simulink model "dynamically_speed_controlled_dc_wound_motor_regen_braking"  (R2025a)
settings: Solver=ode15s  StartTime=0.0  StopTime=40  MaxStep=1e-4  RelTol=1e-3
undefined symbols (not defined in the file): Thyristor
libraries: fl_lib x13, nesl_utility x7, ee_lib x5
(part 1 of 2)
settings Model: Creator=User  LastModifiedBy=User
settings SolverCC: ZeroCrossAlgorithm=Adaptive

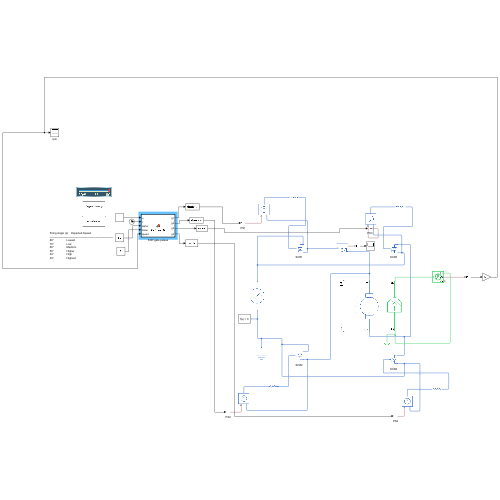
[thumbnail: Simulink's stored preview of the top-level diagram]
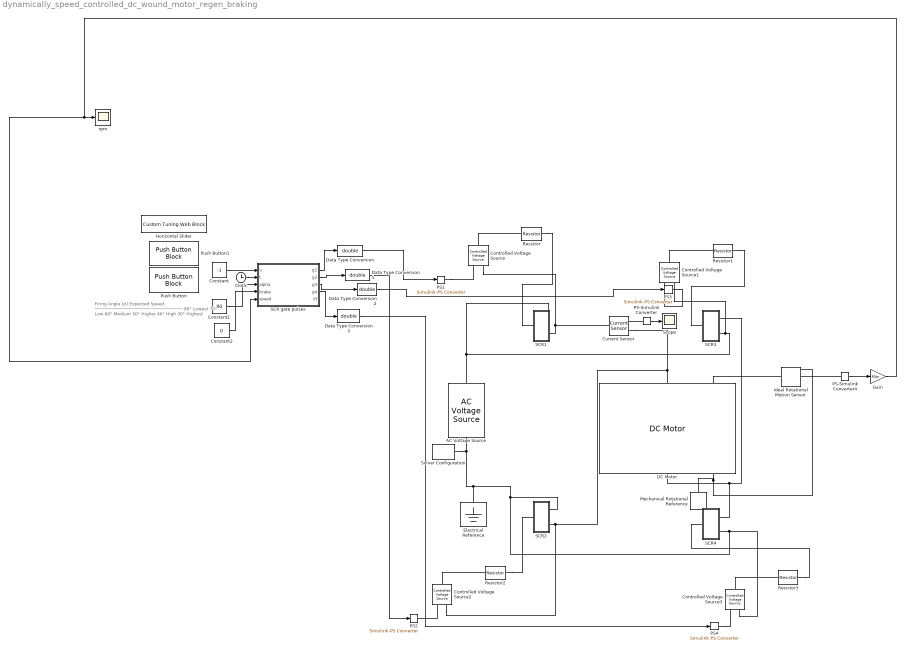
== system dynamically_speed_controlled_dc_wound_motor_regen_braking ==
  note: Firing Angle (α)    Expected Speed
      | ─────────────────────────────────
      | 80°                 Lowest
      | 70°                 Low
      | 60°                 Medium
      | 50°                 Higher
      | 40°                 High
      | 30°                 Highest
  AC Voltage Source : fl_lib/Electrical/Electrical Sources/AC Voltage Source  amp=100 V  shift=0 deg  frequency=50 Hz
  Clock : Clock
  Constant : Constant  Value=-1
  Constant1 : Constant  Value=80
  Constant2 : Constant  Value=0
  Controlled Voltage Source{,1..3} (4 alike) : fl_lib/Electrical/Electrical Sources/Controlled Voltage Source
  Current Sensor : fl_lib/Electrical/Electrical Sensors/Current Sensor
  DC Motor : ee_lib/Electromechanical/Brushed Motors/DC Motor  field_option=ee.enum.field_option.wound  Rf=100 Ohm  Lf=1 H  Laf=0.15 H  If0=0.24 A  parameterization=ee.enum.dcparam_option.circuit_param  Ra=3.9 Ohm  La="0.1  H"  emf_or_torque=ee.enum.emf_or_torque.kv  Kv=0.072e-3 V/rpm  Ki=6.876e-4 N*m/A  T_stall=0.24e-3 N*m  w_max=19100 rpm  w_rated=15000 rpm  P_rated=0.08 W  V_rated=1.5 V  lam_param=ee.enum.lam_param.damping  i_noload=0 A  V_i_noload=1.5 V  J=100 cm^2*g  lam=1e-5 N*m*s/rad  speed0=0 rpm  alpha=3.93e-3 1/K  Tmeas=25 degC  thermal_mass=100 J/K  initial_temperature=25 degC
      settings: InternalSimscapePortConfiguration="{\"Bottom\":[],\"Left\":[{\"id\":\"fp\",\"label\":\"F+\",\"type\":\"foundation.electrical.electrical\"},{\"id\":\"p\",\"label\":\"+\",\"type\":\"foundation.electrical.electrical\"},{\"id\":\"R\",\"label\":\"R\",\"type\":\"foundation.mechanical.rotational.rotational\"}],\"Right\":[{\"id\":\"fn\",\"label\":\"F-\",\"type\":\"foundation.electrical.electrical\"},{\"id\":\"n\",\"label\":\"-\",\"type\":\"foundation.electrical.electrical\"},{\"id\":\"C\",\"label\":\"C\",\"type\":\"foundation.mechanical.rotational.rotational\"}],\"Top\":[]}"
  Data Type Conversion{,1..3} (4 alike) : DataTypeConversion  OutDataTypeStr=double  SaturateOnIntegerOverflow=off  RndMeth=Floor
  Electrical Reference : fl_lib/Electrical/Electrical Elements/Electrical Reference
  Gain : Gain  Gain=30/pi
  Horizontal Slider : CustomTuningWebBlock  LabelPosition=Hide  ShowInitialText=on  Configuration="{\"components\":[{\"name\":\"LinearScaleComponent\",\"settings\":{\"bounds\":{\"max\":80,\"min\":30,\"tickInterval\":\"auto\"},\"internalTickHeightScaleFactor\":0.5,\"labelColor\":[255,255,200],\"labelFont\":{\"font\":\"Arial\",\"fontSize\":12},\"labelOffset\":0.05,\"labelTransparency\":1,\"needleImage\":{\"size\":[596,842],\"src\":\"data:image\\/svg+xml;base64,PD94bWwgdmVyc2lvbj0iMS4wIiBlbmNvZGluZz0idXRmLTgiPz4NCjwhLS0gR2VuZXJhdG9yOiBBZG9iZSBJbGx1c3RyYXRvciAyNS4wLjAsIFNWRyBFeHBvcnQgUGx1Zy1JbiAuIFNWRyBWZXJzaW9uOiA2LjAwIEJ1aWxkIDApICAtLT4NCjxzdmcgdmVyc2lvbj0iMS4xIg0KCSBpZD0ic3ZnOCIgeG1sbnM6Y2M9Imh0dHA6Ly9jcmVhdGl2ZWNvbW1vbnMub3JnL25zIyIgeG1sbnM6ZGM9Imh0dHA6Ly9wdXJsLm9yZy9kYy9lbGVtZW50cy8xLjEvIiB4bWxuczppbmtzY2FwZT0iaHR0cDovL3d3dy5pbmtzY2FwZS5vcmcvbmFtZXNw ...(+2420 chars)\",\"srcOrientation\":\"Right\"},\"needleOffset\":[-0.8044596912521441,-0.0642123287671233],\"needleSize\":{\"height\":0.4337797619047619,\"width\":0.07668067226890757},\"position\":[0.2829861111111111,0.04398634453781513,0.9196428571428571,0.6088789682539683],\"referencePoint\":\"auto\",\"scaleColors\":[],\"scaleColorsSize\":0.2,\"scaleDirection\":\"LR\",\"showLabels\":1,\"showMinorTicks\":0,\"showSpanLine\":1,\"showTicks\":1,\"tickColor\":[252,252,197],\"tickTransparency\":1,\"valueBarColor\":[0,114,189],\"valueBarOffset\":-0.27,\"valueBarSize\":0.1,\"valueBarTransparency\":1}},{\"name\":\"BackgroundImageComponent\",\"settings\":{\"image\":{\"size\":[380,101],\"src\":\"data:image\\/svg+xml;base64,PHN2ZyB4bWxucz0iaHR0cDovL3d3dy53My5vcmcvMjAwMC9zdmciIHhtbG5zOnhsaW5rPSJodHRwOi8vd3d3LnczLm9yZy8xOTk5L3hsaW5rIiB2aWV3Qm94PSIwIDAgMzgwIDEwMSI+PGRlZnM+PHN0eWxlPi5jbHMtMXtmaWxsOiMwMDJiNDI7fS5jbHMtMntmaWxsOiM0MjcwODI7fS5jbHMtM3tmaWxsOnVybCgjcmFkaWFsLWdyYWRpZW50KTt9LmNscy00e2ZpbGw6I2M4YzhjODtzdHJva2U6IzAwMDt9PC9zdHlsZT48cmFkaWFsR3JhZGllbnQgaWQ9InJhZGlhbC1ncmFkaWVudCIgY3g9IjE5MCIgY3k9IjUwLjUiIHI9IjI2OS4yMSIgZ3JhZGllbnRVbml0cz0idXNlclNwYWNlT25Vc2UiPjxzdG9wIG9mZnNldD0iMC4wMSIgc3RvcC1jb2xvcj0iIzNlNGY1OCIvPjxzdG9wIG9mZnNldD0iMC4wNiIgc3RvcC1jb2xvcj0iIzQ0NTc2MSIvPjxzdG9wIG9mZnNldD0iMC4xNSIgc3RvcC1jb2xvcj0iIzU1NmE3NiIvPjxzdG9wIG9mZnNldD0iMC4yNSIgc3RvcC1jb2xvcj0iIzZkODg5NSIvPjxzdG9wIG9mZnNldD0iMC4zOCIgc3RvcC1jb2xvcj0iIzhmYjJjMyIvPjxzdG9wIG9mZnNldD0iMC41MiIgc3RvcC1jb2xvcj0iI2I2ZTRmYSIvPjxzdG9wIG9mZnNldD0iMSIgc3RvcC1jb2xvcj0iIzE1NDY1NyIvPjwvcmFkaWFsR3JhZGllbnQ+PC9kZWZzPjxnIGlkPSJmcmFtZSI+PGcgaWQ9IkxheWVyXzIiIGRhdGEtbmFtZT0iTGF5ZXIgMiI+PGcgaWQ9IkxheWVyXzEtMiIgZGF0YS1uYW1lPSJMYXllciAxLTIiPjxyZWN0IGlkPSJyZWN0MTAzNiIgY2xhc3M9ImNscy0xIiB4PSIxMSIgeT0iMTEiIHdpZHRoPSIzNTgiIGhlaWdodD0iNzkiLz48cGF0aCBpZD0icGF0aDEwMzgiIGNsYXNzPSJjbHMtMiIgZD0iTTgsOFY5M0gzNzJWOFpNMzY5LDkwSDExVjExSDM2OVoiLz48cGF0aCBpZD0icGF0aDEwNDAiIGNsYXNzPSJjbHMtMyIgZD0iTTAsMFYxMDFIMzgwVjBaTTM3Miw5M0g4VjhIMzcyWiIvPjwvZz48L2c+PC9nPjxnIGlkPSJ0cmFjayI+PHBhdGggaWQ9InJlY3QxNjExIiBjbGFzcz0iY2xzLTQiIGQ9Ik0zMy4zNywyNi41OUgzNDYuNjNjNCwwLDcuMjUsMi42LDcuMjUsNS44MWgwYzAsMy4yMS0zLjI1LDUuODItNy4yNSw1LjgySDMzLjM3Yy00LDAtNy4yNS0yLjYxLTcuMjUtNS44MmgwQzI2LjEyLDI5LjE5LDI5LjM3LDI2LjU5LDMzLjM3LDI2LjU5WiIvPjwvZz48L3N2Zz4=\",\"srcOrientation\":\"horizontal\"},\"position\":[0,0,1,1],\"scaleMode\":\"0\"}},{\"name\":\"ForegroundImageComponent\",\"settings\":{\"image\":{\"size\":[0,0],\"src\":\"default\",\"srcOrientation\":[]},\"isForeground\":1,\"position\":[0,0,1,1],\"scaleMode\":\"0\"}}],\"derived\":{\"blockParameters\":{\"ForegroundColor\":[0.9882352941176471,0.9882352941176471,0.7725490196078432],\"Limits\":{\"Max\":80,\"Min\":30,\"Ticks\":\"auto\"},\"ScaleColors\":[],\"ScaleDirection\":\"Clockwise\",\"ScaleMax\":80,\"ScaleMin\":30,\"TickInterval\":\"auto\",\"fixedAspectRatio\":\"on\"}},\"settings\":{\"BindingType\":\"param\",\"aspectRatio\":3.7777777777777777,\"backgroundColor\":[0,0,0,\"1\"],\"backgroundOffset\":0,\"backgroundOpacity\":1,\"fixedAspectRatio\":\"on\",\"foregroundColor\":[252,252,196],\"orientation\":\"horizontal\",\"showBackgroundColor\":false,\"value\":0,\"version\":\"R2023a\"},\"type\":\"LinearGauge\"}"
  Ideal Rotational Motion Sensor : fl_lib/Mechanical/Mechanical Sensors/Ideal Rotational Motion Sensor  reference=foundation.enum.MeasurementReference.difference  acceleration_port=false  velocity_port=true  position_port=true  wrap_angle=false  offset=0 rad
  Mechanical Rotational Reference : fl_lib/Mechanical/Rotational Elements/Mechanical Rotational Reference
  PS-Simulink Converter : nesl_utility/PS-Simulink Converter  PhysicalDomain=network_engine_domain  SubClassName=ps_output  LeftPortType=input  RightPortType=output  PseudoPeriodic=off  Frequencies=[]  VectorFormat=inherit  Unit=A  AffineConversion=off
  PS-Simulink Converter4 : nesl_utility/PS-Simulink Converter  PhysicalDomain=network_engine_domain  SubClassName=ps_output  LeftPortType=input  RightPortType=output  PseudoPeriodic=off  Frequencies=[]  VectorFormat=inherit  Unit=inherit  AffineConversion=off
  PS{1..4} (4 alike) : nesl_utility/Simulink-PS Converter  PhysicalDomain=network_engine_domain  SubClassName=ps_input  LeftPortType=input  RightPortType=output  PseudoPeriodic=off  Frequencies=[]  NoiseDistribution=none  NoiseParameters=[]  Unit=V  AffineConversion=off  FilteringAndDerivatives=provide  SimscapeFilterOrder=1  InputFilterTimeConstant=0.001  UdotUserProvided=0
  Push Button : PushButtonBlock  ButtonText=Accelerator  IconOnColor=[0.0, 0.39215686274509803, 0.0]  IconOffColor=[0.0, 1.0, 0.0]  OffValue=-1.000000
  Push Button1 : PushButtonBlock  ButtonText=Regen Braking  IconOnColor=[0.0, 0.39215686274509803, 0.0]  IconOffColor=[0.0, 1.0, 0.0]  OffValue=0.000000
  Resistor{,1..3} (4 alike) : fl_lib/Electrical/Electrical Elements/Resistor  R=100 Ohm  i_specify=off  i_priority=None  i=0 A  i_nominal_specify=off  i_nominal_value=1  i_nominal_unit=A  v_specify=off  v_priority=None  v=0 V  v_nominal_specify=off  v_nominal_value=1  v_nominal_unit=V
  SCR gate pulses : MATLAB Function  TreatAsAtomicUnit=on
  SCR1 : Subsystem  LoadFcn=ee.selector.SwitchSelectorUtils.forwardingCallback  mask(Semiconductor Switch Selector){SwitchType=Thyristor, LibraryBlockName=Thyristor (Piecewise Linear), ModelingOption=No thermal port, ModelingOptionSSCFile=ee.semiconductors.ideal.thyristor, paramTerminal=Three, port_option=Electrical, CachedInstanceParameters=, FormerSwitchType=Thyristor, FormerLibraryBlockName=Thyristor (Piecewise Linear), FormerModelingOption=No thermal port, CachedSharedParameters={"MOSFET":"{\"port_option\":\"ee.enum.controlport.ps\",\"port_option_unit\":\"1\",\"port_option_conf\":\"compiletime\",\"Ron\":\"0.001\",\"Ron_unit\":\"Ohm\",\"Ron_conf\":\"compiletime\",\"Goff\":\"1e-6\",\"Goff_unit\":\"1/Ohm\",\"Goff_conf\":\"compiletime\",\"Vth\":\"0.5\",\"Vth_unit\":\"V\",\"Vth_conf\":\"compiletime\",\"diode_param\":\"ee.enum.semiconductors.protectionDiode.external\",\"diode_param_unit\":\"1\",\"diode_param_conf\":\"compiletime\",\"diode_Vf\":\"0.8\",\"diode_Vf_unit\":\"V\",\"diode_Vf_conf\":\"compiletime\",\"diode_Ron\":\"0.001\",\"diode_Ron_unit\":\"Ohm\",\"diode_Ron_conf\":\"compiletime\",\"diode_Goff\":\"1e-5\",\"diode_Goff_unit\":\"1/Ohm\",\"diode_Goff_conf\":\"compiletime\",\"diode_C\":\"50e-9\",\"diode_C_unit\":\"F\",\"diode_C_conf\":\"compiletime\",\"diode_iRM\":\"-235\",\"diode_iRM_unit\":\"A\",\"diode_iRM_conf\":\"compiletime\",\"diode_iF\":\"300\",\"diode_iF_unit\":\"A\",\"diode_iF_conf\":\"compiletime\",\"diode_idot\":\"-50\",\"diode_idot_unit\":\"A/us\",\"diode_idot_conf\":\"compiletime\",\"diode_trr_param\":\"ee.enum.converters.diodetrr.trr_factor\",\"diode_trr_param_unit\":\"1\",\"diode_trr_param_conf\":\"compiletime\",\"diode_trr_factor\":\"3\",\"diode_trr_factor_unit\":\"1\",\"diode_trr_factor_conf\":\"compiletime\",\"diode_trr\":\"15\",\"diode_trr_unit\":\"us\",\"diode_trr_conf\":\"compiletime\",\"diode_Qrr\":\"1500\",\"diode_Qrr_unit\":\"s*uA\",\"diode_Qrr_conf\":\"compiletime\"}","IGBT":"","Thyristor":"{\"port_option\":\"ee.enum.controlport.elec\",\"port_option_unit\":\"1\",\"port_option_conf\":\"compiletime\",\"Vf\":\"0.8\",\"Vf_unit\":\"V\",\"Vf_conf\":\"compiletime\",\"Ron\":\"0.001\",\"Ron_unit\":\"Ohm\",\"Ron_conf\":\"compiletime\",\"Goff\":\"1e-5\",\"Goff_unit\":\"1/Ohm\",\"Goff_conf\":\"compiletime\",\"Vgt\":\"6\",\"Vgt_unit\":\"V\",\"Vgt_conf\":\"compiletime\",\"diode_param\":\"ee.enum.semiconductors.protectionDiode.external\",\"diode_param_unit\":\"1\",\"diode_param_conf\":\"compiletime\",\"diode_Vf\":\"0.8\",\"diode_Vf_unit\":\"V\",\"diode_Vf_conf\":\"compiletime\",\"diode_Ron\":\"0.001\",\"diode_Ron_unit\":\"Ohm\",\"diode_Ron_conf\":\"compiletime\",\"diode_Goff\":\"1e-5\",\"diode_Goff_unit\":\"1/Ohm\",\"diode_Goff_conf\":\"compiletime\",\"diode_C\":\"50e-9\",\"diode_C_unit\":\"F\",\"diode_C_conf\":\"compiletime\",\"diode_iRM\":\"-235\",\"diode_iRM_unit\":\"A\",\"diode_iRM_conf\":\"compiletime\",\"diode_iF\":\"300\",\"diode_iF_unit\":\"A\",\"diode_iF_conf\":\"compiletime\",\"diode_idot\":\"-50\",\"diode_idot_unit\":\"A/us\",\"diode_idot_conf\":\"compiletime\",\"diode_trr_param\":\"ee.enum.converters.diodetrr.trr_factor\",\"diode_trr_param_unit\":\"1\",\"diode_trr_param_conf\":\"compiletime\",\"diode_trr_factor\":\"3\",\"diode_trr_factor_unit\":\"1\",\"diode_trr_factor_conf\":\"compiletime\",\"diode_trr\":\"15\",\"diode_trr_unit\":\"us\",\"diode_trr_conf\":\"compiletime\",\"diode_Qrr\":\"1500\",\"diode_Qrr_unit\":\"s*uA\",\"diode_Qrr_conf\":\"compiletime\",\"vak_specify\":\"off\",\"vak_priority\":\"None\",\"vak\":\"0\",\"vak_unit\":\"V\",\"vak_nominal_specify\":\"off\",\"vak_nominal_value\":\"1\",\"vak_nominal_unit\":\"V\",\"vgk_specify\":\"off\",\"vgk_priority\":\"None\",\"vgk\":\"0\",\"vgk_unit\":\"V\",\"vgk_nominal_specify\":\"off\",\"vgk_nominal_value\":\"1\",\"vgk_nominal_unit\":\"V\",\"thermal_loss_option\":\"ee.enum.converters.thermalLossOption.constantvalues\",\"thermal_loss_option_unit\":\"1\",\"thermal_loss_option_conf\":\"compiletime\",\"Von_data\":\"[0, .1, .6, .8, 1, 1.3, 1.6, 2, 2.4; 0, .1, .7, 1, 1.2, 1.5, 1.9, 2.4, 2.8]\",\"Von_data_unit\":\"V\",\"Von_data_conf\":\"compiletime\",\"Tj\":\"[298.15, 398.15]\",\"Tj_unit\":\"K\",\"Tj_conf\":\"compiletime\",\"Iout_data\":\"[0, .1, 1, 5, 10, 20, 40, 70, 100]\",\"Iout_data_unit\":\"A\",\"Iout_data_conf\":\"compiletime\",\"Eon_data\":\"[0, .0024, .024, .12, .2, .48, 1.04, 2.16, 3.24; 0, .003, .03, .15, .25, .6, 1.3, 2.7, 4.05] * 1e-3\",\"Eon_data_unit\":\"J\",\"Eon_data_conf\":\"compiletime\",\"Tj_loss\":\"[298.15, 398.15]\",\"Tj_loss_unit\":\"K\",\"Tj_loss_conf\":\"compiletime\",\"Iout_data_loss\":\"[0, .1, 1, 5, 10, 20, 40, 70, 100]\",\"Iout_data_loss_unit\":\"A\",\"Iout_data_loss_conf\":\"compiletime\",\"Eon_scalar\":\"22.86e-3\",\"Eon_scalar_unit\":\"J\",\"Eon_scalar_conf\":\"compiletime\",\"Eoff_natural_commutation\":\"10e-3\",\"Eoff_natural_commutation_unit\":\"J\",\"Eoff_natural_commutation_conf\":\"compiletime\",\"Voff\":\"300\",\"Voff_unit\":\"V\",\"Voff_conf\":\"compiletime\",\"Iout_scalar\":\"600\",\"Iout_scalar_unit\":\"A\",\"Iout_scalar_conf\":\"compiletime\",\"onCurrentMeasDelay\":\"1e-4\",\"onCurrentMeasDelay_unit\":\"s\",\"onCurrentMeasDelay_conf\":\"compiletime\",\"diodeModelType\":\"ee.enum.converters.diodeModelType.pwl\",\"diodeModelType_unit\":\"1\",\"diodeModelType_conf\":\"compiletime\",\"diodeTableType\":\"ee.enum.diode.tableType.IfMat\",\"diodeTableType_unit\":\"1\",\"diodeTableType_conf\":\"compiletime\",\"diode_IfMat\":\"[.07, .12, .19, 1.75, 4.24, 7.32, 11.2; .16, .3, .72, 2.14, 4.02, 6.35, 9.12]\",\"diode_IfMat_unit\":\"A\",\"diode_IfMat_conf\":\"compiletime\",\"diode_VfMat\":\"[.9, 1.15, 1.25, 1.5, 1.75, 2.17, 2.6, 2.85; .58, .68, .75, 1.1, 1.38, 1.77, 2.27, 2.7]\",\"diode_VfMat_unit\":\"V\",\"diode_VfMat_conf\":\"compiletime\",\"diode_TjVec\":\"[25, 125]\",\"diode_TjVec_unit\":\"degC\",\"diode_TjVec_conf\":\"compiletime\",\"diode_VfVec\":\"[.5, .7, .9, 1.3, 1.7, 2.1, 2.5]\",\"diode_VfVec_unit\":\"V\",\"diode_VfVec_conf\":\"compiletime\",\"diode_IfVec\":\"[.1, .2, .5, 1, 2, 4, 7, 10]\",\"diode_IfVec_unit\":\"A\",\"diode_IfVec_conf\":\"compiletime\",\"diode_rec_loss_model\":\"ee.enum.diode.reverseRecoveryModel.fixed\",\"diode_rec_loss_model_unit\":\"1\",\"diode_rec_loss_model_conf\":\"compiletime\",\"diode_ErecVal\":\"0\",\"diode_ErecVal_unit\":\"J\",\"diode_ErecVal_conf\":\"compiletime\",\"diode_scaleWithIandV\":\"true\",\"diode_scaleWithIandV_unit\":\"1\",\"diode_scaleWithIandV_conf\":\"compiletime\",\"diode_ErecMat\":\"zeros(2, 3)\",\"diode_ErecMat_unit\":\"J\",\"diode_ErecMat_conf\":\"compiletime\",\"diode_TjrecVec\":\"[298.15, 398.15]\",\"diode_TjrecVec_unit\":\"K\",\"diode_TjrecVec_conf\":\"compiletime\",\"diode_IfrecVec\":\"[.1, 1, 10]\",\"diode_IfrecVec_unit\":\"A\",\"diode_IfrecVec_conf\":\"compiletime\",\"diode_IrecVal\":\"10\",\"diode_IrecVal_unit\":\"A\",\"diode_IrecVal_conf\":\"compiletime\",\"diode_VrecVal\":\"10\",\"diode_VrecVal_unit\":\"V\",\"diode_VrecVal_conf\":\"compiletime\",\"diode_tFilter\":\"1 / 1000 / 100\",\"diode_tFilter_unit\":\"s\",\"diode_tFilter_conf\":\"compiletime\",\"thermal_network_parameterization\":\"ee.enum.thermalNetworkTopology.junctionCase\",\"thermal_network_parameterization_unit\":\"1\",\"thermal_network_parameterization_conf\":\"compiletime\",\"Rth\":\"[0, 10]\",\"Rth_unit\":\"K/W\",\"Rth_conf\":\"compiletime\",\"Rth_Cauer\":\"[1, 3, 10]\",\"Rth_Cauer_unit\":\"K/W\",\"Rth_Cauer_conf\":\"compiletime\",\"Rth_Foster\":\"[.08, .14, .22, .16]\",\"Rth_Foster_unit\":\"K/W\",\"Rth_Foster_conf\":\"compiletime\",\"thermal_mass_parameterization\":\"ee.enum.thermalNetwork.timeconstant\",\"thermal_mass_parameterization_unit\":\"1\",\"thermal_mass_parameterization_conf\":\"compiletime\",\"thermal_mass\":\"[0, 1]\",\"thermal_mass_unit\":\"J/K\",\"thermal_mass_conf\":\"compiletime\",\"thermal_mass_Cauer\":\"[.1, .3, 1]\",\"thermal_mass_Cauer_unit\":\"J/K\",\"thermal_mass_Cauer_conf\":\"compiletime\",\"thermal_mass_Foster\":\"[.001, .005, .05, .5]\",\"thermal_mass_Foster_unit\":\"J/K\",\"thermal_mass_Foster_conf\":\"compiletime\",\"thermal_time_constant\":\"[0, 10]\",\"thermal_time_constant_unit\":\"s\",\"thermal_time_constant_conf\":\"compiletime\",\"thermal_time_constant_Cauer\":\"[1, 3, 10]\",\"thermal_time_constant_Cauer_unit\":\"s\",\"thermal_time_constant_Cauer_conf\":\"compiletime\",\"thermal_time_constant_Foster\":\"[7e-05, .0007, .01, .08]\",\"thermal_time_constant_Foster_unit\":\"s\",\"thermal_time_constant_Foster_conf\":\"compiletime\",\"thermal_mass_initial_temperatures\":\"[25, 25]\",\"thermal_mass_initial_temperatures_unit\":\"degC\",\"thermal_mass_initial_temperatures_conf\":\"compiletime\",\"thermal_mass_initial_temperatures_Cauer\":\"[25, 25, 25]\",\"thermal_mass_initial_temperatures_Cauer_unit\":\"degC\",\"thermal_mass_initial_temperatures_Cauer_conf\":\"compiletime\",\"junction_thermal_mass\":\"0.01\",\"junction_thermal_mass_unit\":\"J/K\",\"junction_thermal_mass_conf\":\"compiletime\",\"Tvec_initial_Foster\":\"[25, 25, 25, 25]\",\"Tvec_initial_Foster_unit\":\"degC\",\"Tvec_initial_Foster_conf\":\"compiletime\",\"junction_temperature_specify\":\"off\",\"junction_temperature_priority\":\"None\",\"junction_temperature\":\"25\",\"junction_temperature_unit\":\"degC\",\"junction_temperature_nominal_specify\":\"off\",\"junction_temperature_nominal_value\":\"1\",\"junction_temperature_nominal_unit\":\"degC\",\"Qj_specify\":\"off\",\"Qj_priority\":\"None\",\"Qj\":\"0\",\"Qj_unit\":\"W\",\"Qj_nominal_specify\":\"off\",\"Qj_nominal_value\":\"1\",\"Qj_nominal_unit\":\"W\",\"accumulatedSwitchingLosses_specify\":\"off\",\"accumulatedSwitchingLosses_priority\":\"None\",\"accumulatedSwitchingLosses\":\"0\",\"accumulatedSwitchingLosses_unit\":\"J\",\"i_H\":\"1\",\"i_H_unit\":\"mA\",\"i_H_conf\":\"compiletime\",\"ia\":\"0\",\"ia_unit\":\"A\",\"ia_specify\":\"off\",\"ia_priority\":\"None\",\"ia_nominal_value\":\"1\",\"ia_nominal_unit\":\"A\",\"ia_nominal_specify\":\"off\",\"Gain\":\"10\",\"Gain_conf\":\"compiletime\",\"Gain_unit\":\"1\",\"IDRM\":\"0.01\",\"IDRM_conf\":\"compiletime\",\"IDRM_unit\":\"mA\",\"IT_vec\":\"[.015, .22, .75, 1.4, 2, 2.75, 3.45]\",\"IT_vec_conf\":\"compiletime\",\"IT_vec_unit\":\"A\",\"Q_npn_bc\":\"0\",\"Q_npn_bc_nominal_specify\":\"off\",\"Q_npn_bc_nominal_unit\":\"uC\",\"Q_npn_bc_nominal_value\":\"1\",\"Q_npn_bc_priority\":\"High\",\"Q_npn_bc_specify\":\"off\",\"Q_npn_bc_unit\":\"C\",\"Q_npn_be\":\"0\",\"Q_npn_be_nominal_specify\":\"off\",\"Q_npn_be_nominal_unit\":\"uC\",\"Q_npn_be_nominal_value\":\"1\",\"Q_npn_be_priority\":\"High\",\"Q_npn_be_specify\":\"off\",\"Q_npn_be_unit\":\"C\",\"Q_pnp_be\":\"0\",\"Q_pnp_be_nominal_specify\":\"off\",\"Q_pnp_be_nominal_unit\":\"uC\",\"Q_pnp_be_nominal_value\":\"1\",\"Q_pnp_be_priority\":\"High\",\"Q_pnp_be_specify\":\"off\",\"Q_pnp_be_unit\":\"C\",\"R\":\"120\",\"R_GK\":\"1000\",\"R_GK_conf\":\"compiletime\",\"R_GK_unit\":\"Ohm\",\"R_conf\":\"compiletime\",\"R_unit\":\"Ohm\",\"Rgate\":\"10\",\"Rgate_conf\":\"compiletime\",\"Rgate_unit\":\"Ohm\",\"Rs\":\"87\",\"Rs_conf\":\"compiletime\",\"Rs_unit\":\"kOhm\",\"TF_NPN\":\"0.3\",\"TF_NPN_conf\":\"compiletime\",\"TF_NPN_parameterization\":\"1\",\"TF_NPN_parameterization_conf\":\"compiletime\",\"TF_NPN_parameterization_unit\":\"1\",\"TF_NPN_unit\":\"us\",\"TF_PNP\":\"0.3\",\"TF_PNP_conf\":\"compiletime\",\"TF_PNP_parameterization\":\"1\",\"TF_PNP_parameterization_conf\":\"compiletime\",\"TF_PNP_parameterization_unit\":\"1\",\"TF_PNP_unit\":\"us\",\"T_d\":\"2\",\"T_d_conf\":\"compiletime\",\"T_d_unit\":\"us\",\"Tmeas\":\"25\",\"Tmeas_conf\":\"compiletime\",\"Tmeas_unit\":\"degC\",\"VDRM\":\"400\",\"VDRM_conf\":\"compiletime\",\"VDRM_unit\":\"V\",\"VT_vec\":\"[.75, 1, 1.25, 1.5, 1.75, 2, 2.25]\",\"VT_vec_conf\":\"compiletime\",\"VT_vec_unit\":\"V\",\"V_D\":\"12\",\"V_D_conf\":\"compiletime\",\"V_D_unit\":\"V\",\"dVdt\":\"150\",\"dVdt_conf\":\"compiletime\",\"dVdt_unit\":\"V/us\",\"i_GT\":\"3\",\"i_GT_conf\":\"compiletime\",\"i_GT_unit\":\"uA\",\"i_d\":\"10\",\"i_d_conf\":\"compiletime\",\"i_d_unit\":\"mA\",\"i_on\":\"1\",\"i_on_conf\":\"compiletime\",\"i_on_unit\":\"A\",\"ig\":\"0\",\"ig_nominal_specify\":\"off\",\"ig_nominal_unit\":\"A\",\"ig_nominal_value\":\"1\",\"ig_priority\":\"None\",\"ig_specify\":\"off\",\"ig_unit\":\"A\",\"model_type\":\"ee.enum.semiconductors.thyristorModelType.equations\",\"model_type_conf\":\"compiletime\",\"model_type_unit\":\"1\",\"t_on_curr\":\"1\",\"t_on_curr_conf\":\"compiletime\",\"t_on_curr_unit\":\"mA\",\"t_on_delay\":\"0\",\"t_on_delay_conf\":\"compiletime\",\"t_on_delay_unit\":\"s\",\"t_on_rise\":\"0\",\"t_on_rise_conf\":\"compiletime\",\"t_on_rise_unit\":\"s\",\"v_GT\":\"0.6\",\"v_GT_conf\":\"compiletime\",\"v_GT_unit\":\"V\",\"v_on\":\"1.2\",\"v_on_conf\":\"compiletime\",\"v_on_unit\":\"V\"}","GTO":""}, Version=25.1, SimscapeInternalDisableModelingOption=on}
      mask prompts: SwitchType "physmod:ee:selector:SwitchingDevice"; LibraryBlockName "physmod:ee:selector:LibraryBlock"; ModelingOption "physmod:ee:selector:ModellingOption"; paramTerminal "physmod:ee:selector:Terminals"; port_option "physmod:ee:selector:PortOption"
      mask help: physmod:ee:selector:SemiconductorSwitch_MD
      settings: CopyFcn=ee.selector.SwitchSelectorUtils.copyCallback
      mask Help: web([docroot '/sps/ref/semiconductorswitchselector.html'])
      mask TypeOptions SwitchType: physmod:ee:selector:MOSFET_PV | physmod:ee:selector:IGBT_PV | physmod:ee:selector:Thyristor_PV | physmod:ee:selector:GTO_PV
      mask Callback SwitchType: ee.selector.SwitchSelectorUtils.selectSwitch
      mask TypeOptions LibraryBlockName: Thyristor | Thyristor (Piecewise Linear)
      mask Callback LibraryBlockName: ee.selector.SwitchSelectorUtils.selectSwitch
      mask TypeOptions ModelingOption: No thermal port | Show thermal port
      mask Callback ModelingOption: ee.selector.SwitchSelectorUtils.selectSwitch
      mask TypeOptions paramTerminal: physmod:ee:library:comments:enum:mosfet:numberOfTerminals:map_Three | physmod:ee:library:comments:enum:mosfet:numberOfTerminals:map_Four
      mask Callback paramTerminal: ee.selector.SwitchSelectorUtils.addOrRemoveFourthPort
      mask TypeOptions port_option: physmod:ee:library:comments:enum:controlport:map_PS | physmod:ee:library:comments:enum:controlport:map_Electrical
      mask Callback port_option: ee.selector.SwitchSelectorUtils.updatePortOption
      mask DialogControl DropdownsTab Prompt: physmod:ee:selector:SwitchSelection
      mask DialogControl SwitchType Prompt: Switching device
      mask DialogControl LibraryBlockName Prompt: Library block
      mask DialogControl ModelingOption Prompt: Modeling option
      mask DialogControl paramTerminal Prompt: Number of terminals
      mask DialogControl port_option Prompt: Gate-control port
      mask DialogControl ConfigureSwitchButton Prompt: physmod:ee:selector:EditParams
      mask DialogControl ConfigureSwitchButton Callback: ee.selector.SwitchSelectorUtils.openSwitchBlock
      mask DialogControl SwitchDescription Prompt: physmod:ee:library:comments:semiconductors:ideal:thyristor:Description
      mask DialogControl RemoveMask Prompt: physmod:ee:selector:RemoveMask
      mask DialogControl RemoveMask Callback: ee.selector.SwitchSelectorUtils.removeMask
  SCR2 : Subsystem  LoadFcn=ee.selector.SwitchSelectorUtils.forwardingCallback  mask(Semiconductor Switch Selector){SwitchType=Thyristor, LibraryBlockName=Thyristor (Piecewise Linear), ModelingOption=No thermal port, ModelingOptionSSCFile=ee.semiconductors.ideal.thyristor, paramTerminal=Three, port_option=Electrical, CachedInstanceParameters=, FormerSwitchType=Thyristor, FormerLibraryBlockName=Thyristor (Piecewise Linear), FormerModelingOption=No thermal port, CachedSharedParameters={"MOSFET":"{\"port_option\":\"ee.enum.controlport.ps\",\"port_option_unit\":\"1\",\"port_option_conf\":\"compiletime\",\"Ron\":\"0.001\",\"Ron_unit\":\"Ohm\",\"Ron_conf\":\"compiletime\",\"Goff\":\"1e-6\",\"Goff_unit\":\"1/Ohm\",\"Goff_conf\":\"compiletime\",\"Vth\":\"0.5\",\"Vth_unit\":\"V\",\"Vth_conf\":\"compiletime\",\"diode_param\":\"ee.enum.semiconductors.protectionDiode.external\",\"diode_param_unit\":\"1\",\"diode_param_conf\":\"compiletime\",\"diode_Vf\":\"0.8\",\"diode_Vf_unit\":\"V\",\"diode_Vf_conf\":\"compiletime\",\"diode_Ron\":\"0.001\",\"diode_Ron_unit\":\"Ohm\",\"diode_Ron_conf\":\"compiletime\",\"diode_Goff\":\"1e-5\",\"diode_Goff_unit\":\"1/Ohm\",\"diode_Goff_conf\":\"compiletime\",\"diode_C\":\"50e-9\",\"diode_C_unit\":\"F\",\"diode_C_conf\":\"compiletime\",\"diode_iRM\":\"-235\",\"diode_iRM_unit\":\"A\",\"diode_iRM_conf\":\"compiletime\",\"diode_iF\":\"300\",\"diode_iF_unit\":\"A\",\"diode_iF_conf\":\"compiletime\",\"diode_idot\":\"-50\",\"diode_idot_unit\":\"A/us\",\"diode_idot_conf\":\"compiletime\",\"diode_trr_param\":\"ee.enum.converters.diodetrr.trr_factor\",\"diode_trr_param_unit\":\"1\",\"diode_trr_param_conf\":\"compiletime\",\"diode_trr_factor\":\"3\",\"diode_trr_factor_unit\":\"1\",\"diode_trr_factor_conf\":\"compiletime\",\"diode_trr\":\"15\",\"diode_trr_unit\":\"us\",\"diode_trr_conf\":\"compiletime\",\"diode_Qrr\":\"1500\",\"diode_Qrr_unit\":\"s*uA\",\"diode_Qrr_conf\":\"compiletime\"}","IGBT":"","Thyristor":"{\"port_option\":\"ee.enum.controlport.elec\",\"port_option_unit\":\"1\",\"port_option_conf\":\"compiletime\",\"Vf\":\"0.8\",\"Vf_unit\":\"V\",\"Vf_conf\":\"compiletime\",\"Ron\":\"0.001\",\"Ron_unit\":\"Ohm\",\"Ron_conf\":\"compiletime\",\"Goff\":\"1e-5\",\"Goff_unit\":\"1/Ohm\",\"Goff_conf\":\"compiletime\",\"Vgt\":\"6\",\"Vgt_unit\":\"V\",\"Vgt_conf\":\"compiletime\",\"diode_param\":\"ee.enum.semiconductors.protectionDiode.external\",\"diode_param_unit\":\"1\",\"diode_param_conf\":\"compiletime\",\"diode_Vf\":\"0.8\",\"diode_Vf_unit\":\"V\",\"diode_Vf_conf\":\"compiletime\",\"diode_Ron\":\"0.001\",\"diode_Ron_unit\":\"Ohm\",\"diode_Ron_conf\":\"compiletime\",\"diode_Goff\":\"1e-5\",\"diode_Goff_unit\":\"1/Ohm\",\"diode_Goff_conf\":\"compiletime\",\"diode_C\":\"50e-9\",\"diode_C_unit\":\"F\",\"diode_C_conf\":\"compiletime\",\"diode_iRM\":\"-235\",\"diode_iRM_unit\":\"A\",\"diode_iRM_conf\":\"compiletime\",\"diode_iF\":\"300\",\"diode_iF_unit\":\"A\",\"diode_iF_conf\":\"compiletime\",\"diode_idot\":\"-50\",\"diode_idot_unit\":\"A/us\",\"diode_idot_conf\":\"compiletime\",\"diode_trr_param\":\"ee.enum.converters.diodetrr.trr_factor\",\"diode_trr_param_unit\":\"1\",\"diode_trr_param_conf\":\"compiletime\",\"diode_trr_factor\":\"3\",\"diode_trr_factor_unit\":\"1\",\"diode_trr_factor_conf\":\"compiletime\",\"diode_trr\":\"15\",\"diode_trr_unit\":\"us\",\"diode_trr_conf\":\"compiletime\",\"diode_Qrr\":\"1500\",\"diode_Qrr_unit\":\"s*uA\",\"diode_Qrr_conf\":\"compiletime\",\"vak_specify\":\"off\",\"vak_priority\":\"None\",\"vak\":\"0\",\"vak_unit\":\"V\",\"vak_nominal_specify\":\"off\",\"vak_nominal_value\":\"1\",\"vak_nominal_unit\":\"V\",\"vgk_specify\":\"off\",\"vgk_priority\":\"None\",\"vgk\":\"0\",\"vgk_unit\":\"V\",\"vgk_nominal_specify\":\"off\",\"vgk_nominal_value\":\"1\",\"vgk_nominal_unit\":\"V\",\"thermal_loss_option\":\"ee.enum.converters.thermalLossOption.constantvalues\",\"thermal_loss_option_unit\":\"1\",\"thermal_loss_option_conf\":\"compiletime\",\"Von_data\":\"[0, .1, .6, .8, 1, 1.3, 1.6, 2, 2.4; 0, .1, .7, 1, 1.2, 1.5, 1.9, 2.4, 2.8]\",\"Von_data_unit\":\"V\",\"Von_data_conf\":\"compiletime\",\"Tj\":\"[298.15, 398.15]\",\"Tj_unit\":\"K\",\"Tj_conf\":\"compiletime\",\"Iout_data\":\"[0, .1, 1, 5, 10, 20, 40, 70, 100]\",\"Iout_data_unit\":\"A\",\"Iout_data_conf\":\"compiletime\",\"Eon_data\":\"[0, .0024, .024, .12, .2, .48, 1.04, 2.16, 3.24; 0, .003, .03, .15, .25, .6, 1.3, 2.7, 4.05] * 1e-3\",\"Eon_data_unit\":\"J\",\"Eon_data_conf\":\"compiletime\",\"Tj_loss\":\"[298.15, 398.15]\",\"Tj_loss_unit\":\"K\",\"Tj_loss_conf\":\"compiletime\",\"Iout_data_loss\":\"[0, .1, 1, 5, 10, 20, 40, 70, 100]\",\"Iout_data_loss_unit\":\"A\",\"Iout_data_loss_conf\":\"compiletime\",\"Eon_scalar\":\"22.86e-3\",\"Eon_scalar_unit\":\"J\",\"Eon_scalar_conf\":\"compiletime\",\"Eoff_natural_commutation\":\"10e-3\",\"Eoff_natural_commutation_unit\":\"J\",\"Eoff_natural_commutation_conf\":\"compiletime\",\"Voff\":\"300\",\"Voff_unit\":\"V\",\"Voff_conf\":\"compiletime\",\"Iout_scalar\":\"600\",\"Iout_scalar_unit\":\"A\",\"Iout_scalar_conf\":\"compiletime\",\"onCurrentMeasDelay\":\"1e-4\",\"onCurrentMeasDelay_unit\":\"s\",\"onCurrentMeasDelay_conf\":\"compiletime\",\"diodeModelType\":\"ee.enum.converters.diodeModelType.pwl\",\"diodeModelType_unit\":\"1\",\"diodeModelType_conf\":\"compiletime\",\"diodeTableType\":\"ee.enum.diode.tableType.IfMat\",\"diodeTableType_unit\":\"1\",\"diodeTableType_conf\":\"compiletime\",\"diode_IfMat\":\"[.07, .12, .19, 1.75, 4.24, 7.32, 11.2; .16, .3, .72, 2.14, 4.02, 6.35, 9.12]\",\"diode_IfMat_unit\":\"A\",\"diode_IfMat_conf\":\"compiletime\",\"diode_VfMat\":\"[.9, 1.15, 1.25, 1.5, 1.75, 2.17, 2.6, 2.85; .58, .68, .75, 1.1, 1.38, 1.77, 2.27, 2.7]\",\"diode_VfMat_unit\":\"V\",\"diode_VfMat_conf\":\"compiletime\",\"diode_TjVec\":\"[25, 125]\",\"diode_TjVec_unit\":\"degC\",\"diode_TjVec_conf\":\"compiletime\",\"diode_VfVec\":\"[.5, .7, .9, 1.3, 1.7, 2.1, 2.5]\",\"diode_VfVec_unit\":\"V\",\"diode_VfVec_conf\":\"compiletime\",\"diode_IfVec\":\"[.1, .2, .5, 1, 2, 4, 7, 10]\",\"diode_IfVec_unit\":\"A\",\"diode_IfVec_conf\":\"compiletime\",\"diode_rec_loss_model\":\"ee.enum.diode.reverseRecoveryModel.fixed\",\"diode_rec_loss_model_unit\":\"1\",\"diode_rec_loss_model_conf\":\"compiletime\",\"diode_ErecVal\":\"0\",\"diode_ErecVal_unit\":\"J\",\"diode_ErecVal_conf\":\"compiletime\",\"diode_scaleWithIandV\":\"true\",\"diode_scaleWithIandV_unit\":\"1\",\"diode_scaleWithIandV_conf\":\"compiletime\",\"diode_ErecMat\":\"zeros(2, 3)\",\"diode_ErecMat_unit\":\"J\",\"diode_ErecMat_conf\":\"compiletime\",\"diode_TjrecVec\":\"[298.15, 398.15]\",\"diode_TjrecVec_unit\":\"K\",\"diode_TjrecVec_conf\":\"compiletime\",\"diode_IfrecVec\":\"[.1, 1, 10]\",\"diode_IfrecVec_unit\":\"A\",\"diode_IfrecVec_conf\":\"compiletime\",\"diode_IrecVal\":\"10\",\"diode_IrecVal_unit\":\"A\",\"diode_IrecVal_conf\":\"compiletime\",\"diode_VrecVal\":\"10\",\"diode_VrecVal_unit\":\"V\",\"diode_VrecVal_conf\":\"compiletime\",\"diode_tFilter\":\"1 / 1000 / 100\",\"diode_tFilter_unit\":\"s\",\"diode_tFilter_conf\":\"compiletime\",\"thermal_network_parameterization\":\"ee.enum.thermalNetworkTopology.junctionCase\",\"thermal_network_parameterization_unit\":\"1\",\"thermal_network_parameterization_conf\":\"compiletime\",\"Rth\":\"[0, 10]\",\"Rth_unit\":\"K/W\",\"Rth_conf\":\"compiletime\",\"Rth_Cauer\":\"[1, 3, 10]\",\"Rth_Cauer_unit\":\"K/W\",\"Rth_Cauer_conf\":\"compiletime\",\"Rth_Foster\":\"[.08, .14, .22, .16]\",\"Rth_Foster_unit\":\"K/W\",\"Rth_Foster_conf\":\"compiletime\",\"thermal_mass_parameterization\":\"ee.enum.thermalNetwork.timeconstant\",\"thermal_mass_parameterization_unit\":\"1\",\"thermal_mass_parameterization_conf\":\"compiletime\",\"thermal_mass\":\"[0, 1]\",\"thermal_mass_unit\":\"J/K\",\"thermal_mass_conf\":\"compiletime\",\"thermal_mass_Cauer\":\"[.1, .3, 1]\",\"thermal_mass_Cauer_unit\":\"J/K\",\"thermal_mass_Cauer_conf\":\"compiletime\",\"thermal_mass_Foster\":\"[.001, .005, .05, .5]\",\"thermal_mass_Foster_unit\":\"J/K\",\"thermal_mass_Foster_conf\":\"compiletime\",\"thermal_time_constant\":\"[0, 10]\",\"thermal_time_constant_unit\":\"s\",\"thermal_time_constant_conf\":\"compiletime\",\"thermal_time_constant_Cauer\":\"[1, 3, 10]\",\"thermal_time_constant_Cauer_unit\":\"s\",\"thermal_time_constant_Cauer_conf\":\"compiletime\",\"thermal_time_constant_Foster\":\"[7e-05, .0007, .01, .08]\",\"thermal_time_constant_Foster_unit\":\"s\",\"thermal_time_constant_Foster_conf\":\"compiletime\",\"thermal_mass_initial_temperatures\":\"[25, 25]\",\"thermal_mass_initial_temperatures_unit\":\"degC\",\"thermal_mass_initial_temperatures_conf\":\"compiletime\",\"thermal_mass_initial_temperatures_Cauer\":\"[25, 25, 25]\",\"thermal_mass_initial_temperatures_Cauer_unit\":\"degC\",\"thermal_mass_initial_temperatures_Cauer_conf\":\"compiletime\",\"junction_thermal_mass\":\"0.01\",\"junction_thermal_mass_unit\":\"J/K\",\"junction_thermal_mass_conf\":\"compiletime\",\"Tvec_initial_Foster\":\"[25, 25, 25, 25]\",\"Tvec_initial_Foster_unit\":\"degC\",\"Tvec_initial_Foster_conf\":\"compiletime\",\"junction_temperature_specify\":\"off\",\"junction_temperature_priority\":\"None\",\"junction_temperature\":\"25\",\"junction_temperature_unit\":\"degC\",\"junction_temperature_nominal_specify\":\"off\",\"junction_temperature_nominal_value\":\"1\",\"junction_temperature_nominal_unit\":\"degC\",\"Qj_specify\":\"off\",\"Qj_priority\":\"None\",\"Qj\":\"0\",\"Qj_unit\":\"W\",\"Qj_nominal_specify\":\"off\",\"Qj_nominal_value\":\"1\",\"Qj_nominal_unit\":\"W\",\"accumulatedSwitchingLosses_specify\":\"off\",\"accumulatedSwitchingLosses_priority\":\"None\",\"accumulatedSwitchingLosses\":\"0\",\"accumulatedSwitchingLosses_unit\":\"J\",\"i_H\":\"1\",\"i_H_unit\":\"mA\",\"i_H_conf\":\"compiletime\",\"ia\":\"0\",\"ia_unit\":\"A\",\"ia_specify\":\"off\",\"ia_priority\":\"None\",\"ia_nominal_value\":\"1\",\"ia_nominal_unit\":\"A\",\"ia_nominal_specify\":\"off\",\"Gain\":\"10\",\"Gain_conf\":\"compiletime\",\"Gain_unit\":\"1\",\"IDRM\":\"0.01\",\"IDRM_conf\":\"compiletime\",\"IDRM_unit\":\"mA\",\"IT_vec\":\"[.015, .22, .75, 1.4, 2, 2.75, 3.45]\",\"IT_vec_conf\":\"compiletime\",\"IT_vec_unit\":\"A\",\"Q_npn_bc\":\"0\",\"Q_npn_bc_nominal_specify\":\"off\",\"Q_npn_bc_nominal_unit\":\"uC\",\"Q_npn_bc_nominal_value\":\"1\",\"Q_npn_bc_priority\":\"High\",\"Q_npn_bc_specify\":\"off\",\"Q_npn_bc_unit\":\"C\",\"Q_npn_be\":\"0\",\"Q_npn_be_nominal_specify\":\"off\",\"Q_npn_be_nominal_unit\":\"uC\",\"Q_npn_be_nominal_value\":\"1\",\"Q_npn_be_priority\":\"High\",\"Q_npn_be_specify\":\"off\",\"Q_npn_be_unit\":\"C\",\"Q_pnp_be\":\"0\",\"Q_pnp_be_nominal_specify\":\"off\",\"Q_pnp_be_nominal_unit\":\"uC\",\"Q_pnp_be_nominal_value\":\"1\",\"Q_pnp_be_priority\":\"High\",\"Q_pnp_be_specify\":\"off\",\"Q_pnp_be_unit\":\"C\",\"R\":\"120\",\"R_GK\":\"1000\",\"R_GK_conf\":\"compiletime\",\"R_GK_unit\":\"Ohm\",\"R_conf\":\"compiletime\",\"R_unit\":\"Ohm\",\"Rgate\":\"10\",\"Rgate_conf\":\"compiletime\",\"Rgate_unit\":\"Ohm\",\"Rs\":\"87\",\"Rs_conf\":\"compiletime\",\"Rs_unit\":\"kOhm\",\"TF_NPN\":\"0.3\",\"TF_NPN_conf\":\"compiletime\",\"TF_NPN_parameterization\":\"1\",\"TF_NPN_parameterization_conf\":\"compiletime\",\"TF_NPN_parameterization_unit\":\"1\",\"TF_NPN_unit\":\"us\",\"TF_PNP\":\"0.3\",\"TF_PNP_conf\":\"compiletime\",\"TF_PNP_parameterization\":\"1\",\"TF_PNP_parameterization_conf\":\"compiletime\",\"TF_PNP_parameterization_unit\":\"1\",\"TF_PNP_unit\":\"us\",\"T_d\":\"2\",\"T_d_conf\":\"compiletime\",\"T_d_unit\":\"us\",\"Tmeas\":\"25\",\"Tmeas_conf\":\"compiletime\",\"Tmeas_unit\":\"degC\",\"VDRM\":\"400\",\"VDRM_conf\":\"compiletime\",\"VDRM_unit\":\"V\",\"VT_vec\":\"[.75, 1, 1.25, 1.5, 1.75, 2, 2.25]\",\"VT_vec_conf\":\"compiletime\",\"VT_vec_unit\":\"V\",\"V_D\":\"12\",\"V_D_conf\":\"compiletime\",\"V_D_unit\":\"V\",\"dVdt\":\"150\",\"dVdt_conf\":\"compiletime\",\"dVdt_unit\":\"V/us\",\"i_GT\":\"3\",\"i_GT_conf\":\"compiletime\",\"i_GT_unit\":\"uA\",\"i_d\":\"10\",\"i_d_conf\":\"compiletime\",\"i_d_unit\":\"mA\",\"i_on\":\"1\",\"i_on_conf\":\"compiletime\",\"i_on_unit\":\"A\",\"ig\":\"0\",\"ig_nominal_specify\":\"off\",\"ig_nominal_unit\":\"A\",\"ig_nominal_value\":\"1\",\"ig_priority\":\"None\",\"ig_specify\":\"off\",\"ig_unit\":\"A\",\"model_type\":\"ee.enum.semiconductors.thyristorModelType.equations\",\"model_type_conf\":\"compiletime\",\"model_type_unit\":\"1\",\"t_on_curr\":\"1\",\"t_on_curr_conf\":\"compiletime\",\"t_on_curr_unit\":\"mA\",\"t_on_delay\":\"0\",\"t_on_delay_conf\":\"compiletime\",\"t_on_delay_unit\":\"s\",\"t_on_rise\":\"0\",\"t_on_rise_conf\":\"compiletime\",\"t_on_rise_unit\":\"s\",\"v_GT\":\"0.6\",\"v_GT_conf\":\"compiletime\",\"v_GT_unit\":\"V\",\"v_on\":\"1.2\",\"v_on_conf\":\"compiletime\",\"v_on_unit\":\"V\"}","GTO":""}, Version=25.1, SimscapeInternalDisableModelingOption=on}
      mask prompts: SwitchType "physmod:ee:selector:SwitchingDevice"; LibraryBlockName "physmod:ee:selector:LibraryBlock"; ModelingOption "physmod:ee:selector:ModellingOption"; paramTerminal "physmod:ee:selector:Terminals"; port_option "physmod:ee:selector:PortOption"
      mask help: physmod:ee:selector:SemiconductorSwitch_MD
      settings: CopyFcn=ee.selector.SwitchSelectorUtils.copyCallback
      mask Help: web([docroot '/sps/ref/semiconductorswitchselector.html'])
      mask TypeOptions SwitchType: physmod:ee:selector:MOSFET_PV | physmod:ee:selector:IGBT_PV | physmod:ee:selector:Thyristor_PV | physmod:ee:selector:GTO_PV
      mask Callback SwitchType: ee.selector.SwitchSelectorUtils.selectSwitch
      mask TypeOptions LibraryBlockName: Thyristor | Thyristor (Piecewise Linear)
      mask Callback LibraryBlockName: ee.selector.SwitchSelectorUtils.selectSwitch
      mask TypeOptions ModelingOption: No thermal port | Show thermal port
      mask Callback ModelingOption: ee.selector.SwitchSelectorUtils.selectSwitch
      mask TypeOptions paramTerminal: physmod:ee:library:comments:enum:mosfet:numberOfTerminals:map_Three | physmod:ee:library:comments:enum:mosfet:numberOfTerminals:map_Four
      mask Callback paramTerminal: ee.selector.SwitchSelectorUtils.addOrRemoveFourthPort
      mask TypeOptions port_option: physmod:ee:library:comments:enum:controlport:map_PS | physmod:ee:library:comments:enum:controlport:map_Electrical
      mask Callback port_option: ee.selector.SwitchSelectorUtils.updatePortOption
      mask DialogControl DropdownsTab Prompt: physmod:ee:selector:SwitchSelection
      mask DialogControl SwitchType Prompt: Switching device
      mask DialogControl LibraryBlockName Prompt: Library block
      mask DialogControl ModelingOption Prompt: Modeling option
      mask DialogControl paramTerminal Prompt: Number of terminals
      mask DialogControl port_option Prompt: Gate-control port
      mask DialogControl ConfigureSwitchButton Prompt: physmod:ee:selector:EditParams
      mask DialogControl ConfigureSwitchButton Callback: ee.selector.SwitchSelectorUtils.openSwitchBlock
      mask DialogControl SwitchDescription Prompt: physmod:ee:library:comments:semiconductors:ideal:thyristor:Description
      mask DialogControl RemoveMask Prompt: physmod:ee:selector:RemoveMask
      mask DialogControl RemoveMask Callback: ee.selector.SwitchSelectorUtils.removeMask
  SCR3 : Subsystem  LoadFcn=ee.selector.SwitchSelectorUtils.forwardingCallback  mask(Semiconductor Switch Selector){SwitchType=Thyristor, LibraryBlockName=Thyristor (Piecewise Linear), ModelingOption=No thermal port, ModelingOptionSSCFile=ee.semiconductors.ideal.thyristor, paramTerminal=Three, port_option=Electrical, CachedInstanceParameters=, FormerSwitchType=Thyristor, FormerLibraryBlockName=Thyristor (Piecewise Linear), FormerModelingOption=No thermal port, CachedSharedParameters={"MOSFET":"{\"port_option\":\"ee.enum.controlport.ps\",\"port_option_unit\":\"1\",\"port_option_conf\":\"compiletime\",\"Ron\":\"0.001\",\"Ron_unit\":\"Ohm\",\"Ron_conf\":\"compiletime\",\"Goff\":\"1e-6\",\"Goff_unit\":\"1/Ohm\",\"Goff_conf\":\"compiletime\",\"Vth\":\"0.5\",\"Vth_unit\":\"V\",\"Vth_conf\":\"compiletime\",\"diode_param\":\"ee.enum.semiconductors.protectionDiode.external\",\"diode_param_unit\":\"1\",\"diode_param_conf\":\"compiletime\",\"diode_Vf\":\"0.8\",\"diode_Vf_unit\":\"V\",\"diode_Vf_conf\":\"compiletime\",\"diode_Ron\":\"0.001\",\"diode_Ron_unit\":\"Ohm\",\"diode_Ron_conf\":\"compiletime\",\"diode_Goff\":\"1e-5\",\"diode_Goff_unit\":\"1/Ohm\",\"diode_Goff_conf\":\"compiletime\",\"diode_C\":\"50e-9\",\"diode_C_unit\":\"F\",\"diode_C_conf\":\"compiletime\",\"diode_iRM\":\"-235\",\"diode_iRM_unit\":\"A\",\"diode_iRM_conf\":\"compiletime\",\"diode_iF\":\"300\",\"diode_iF_unit\":\"A\",\"diode_iF_conf\":\"compiletime\",\"diode_idot\":\"-50\",\"diode_idot_unit\":\"A/us\",\"diode_idot_conf\":\"compiletime\",\"diode_trr_param\":\"ee.enum.converters.diodetrr.trr_factor\",\"diode_trr_param_unit\":\"1\",\"diode_trr_param_conf\":\"compiletime\",\"diode_trr_factor\":\"3\",\"diode_trr_factor_unit\":\"1\",\"diode_trr_factor_conf\":\"compiletime\",\"diode_trr\":\"15\",\"diode_trr_unit\":\"us\",\"diode_trr_conf\":\"compiletime\",\"diode_Qrr\":\"1500\",\"diode_Qrr_unit\":\"s*uA\",\"diode_Qrr_conf\":\"compiletime\"}","IGBT":"","Thyristor":"{\"port_option\":\"ee.enum.controlport.elec\",\"port_option_unit\":\"1\",\"port_option_conf\":\"compiletime\",\"Vf\":\"0.8\",\"Vf_unit\":\"V\",\"Vf_conf\":\"compiletime\",\"Ron\":\"0.001\",\"Ron_unit\":\"Ohm\",\"Ron_conf\":\"compiletime\",\"Goff\":\"1e-5\",\"Goff_unit\":\"1/Ohm\",\"Goff_conf\":\"compiletime\",\"Vgt\":\"6\",\"Vgt_unit\":\"V\",\"Vgt_conf\":\"compiletime\",\"diode_param\":\"ee.enum.semiconductors.protectionDiode.external\",\"diode_param_unit\":\"1\",\"diode_param_conf\":\"compiletime\",\"diode_Vf\":\"0.8\",\"diode_Vf_unit\":\"V\",\"diode_Vf_conf\":\"compiletime\",\"diode_Ron\":\"0.001\",\"diode_Ron_unit\":\"Ohm\",\"diode_Ron_conf\":\"compiletime\",\"diode_Goff\":\"1e-5\",\"diode_Goff_unit\":\"1/Ohm\",\"diode_Goff_conf\":\"compiletime\",\"diode_C\":\"50e-9\",\"diode_C_unit\":\"F\",\"diode_C_conf\":\"compiletime\",\"diode_iRM\":\"-235\",\"diode_iRM_unit\":\"A\",\"diode_iRM_conf\":\"compiletime\",\"diode_iF\":\"300\",\"diode_iF_unit\":\"A\",\"diode_iF_conf\":\"compiletime\",\"diode_idot\":\"-50\",\"diode_idot_unit\":\"A/us\",\"diode_idot_conf\":\"compiletime\",\"diode_trr_param\":\"ee.enum.converters.diodetrr.trr_factor\",\"diode_trr_param_unit\":\"1\",\"diode_trr_param_conf\":\"compiletime\",\"diode_trr_factor\":\"3\",\"diode_trr_factor_unit\":\"1\",\"diode_trr_factor_conf\":\"compiletime\",\"diode_trr\":\"15\",\"diode_trr_unit\":\"us\",\"diode_trr_conf\":\"compiletime\",\"diode_Qrr\":\"1500\",\"diode_Qrr_unit\":\"s*uA\",\"diode_Qrr_conf\":\"compiletime\",\"vak_specify\":\"off\",\"vak_priority\":\"None\",\"vak\":\"0\",\"vak_unit\":\"V\",\"vak_nominal_specify\":\"off\",\"vak_nominal_value\":\"1\",\"vak_nominal_unit\":\"V\",\"vgk_specify\":\"off\",\"vgk_priority\":\"None\",\"vgk\":\"0\",\"vgk_unit\":\"V\",\"vgk_nominal_specify\":\"off\",\"vgk_nominal_value\":\"1\",\"vgk_nominal_unit\":\"V\",\"thermal_loss_option\":\"ee.enum.converters.thermalLossOption.constantvalues\",\"thermal_loss_option_unit\":\"1\",\"thermal_loss_option_conf\":\"compiletime\",\"Von_data\":\"[0, .1, .6, .8, 1, 1.3, 1.6, 2, 2.4; 0, .1, .7, 1, 1.2, 1.5, 1.9, 2.4, 2.8]\",\"Von_data_unit\":\"V\",\"Von_data_conf\":\"compiletime\",\"Tj\":\"[298.15, 398.15]\",\"Tj_unit\":\"K\",\"Tj_conf\":\"compiletime\",\"Iout_data\":\"[0, .1, 1, 5, 10, 20, 40, 70, 100]\",\"Iout_data_unit\":\"A\",\"Iout_data_conf\":\"compiletime\",\"Eon_data\":\"[0, .0024, .024, .12, .2, .48, 1.04, 2.16, 3.24; 0, .003, .03, .15, .25, .6, 1.3, 2.7, 4.05] * 1e-3\",\"Eon_data_unit\":\"J\",\"Eon_data_conf\":\"compiletime\",\"Tj_loss\":\"[298.15, 398.15]\",\"Tj_loss_unit\":\"K\",\"Tj_loss_conf\":\"compiletime\",\"Iout_data_loss\":\"[0, .1, 1, 5, 10, 20, 40, 70, 100]\",\"Iout_data_loss_unit\":\"A\",\"Iout_data_loss_conf\":\"compiletime\",\"Eon_scalar\":\"22.86e-3\",\"Eon_scalar_unit\":\"J\",\"Eon_scalar_conf\":\"compiletime\",\"Eoff_natural_commutation\":\"10e-3\",\"Eoff_natural_commutation_unit\":\"J\",\"Eoff_natural_commutation_conf\":\"compiletime\",\"Voff\":\"300\",\"Voff_unit\":\"V\",\"Voff_conf\":\"compiletime\",\"Iout_scalar\":\"600\",\"Iout_scalar_unit\":\"A\",\"Iout_scalar_conf\":\"compiletime\",\"onCurrentMeasDelay\":\"1e-4\",\"onCurrentMeasDelay_unit\":\"s\",\"onCurrentMeasDelay_conf\":\"compiletime\",\"diodeModelType\":\"ee.enum.converters.diodeModelType.pwl\",\"diodeModelType_unit\":\"1\",\"diodeModelType_conf\":\"compiletime\",\"diodeTableType\":\"ee.enum.diode.tableType.IfMat\",\"diodeTableType_unit\":\"1\",\"diodeTableType_conf\":\"compiletime\",\"diode_IfMat\":\"[.07, .12, .19, 1.75, 4.24, 7.32, 11.2; .16, .3, .72, 2.14, 4.02, 6.35, 9.12]\",\"diode_IfMat_unit\":\"A\",\"diode_IfMat_conf\":\"compiletime\",\"diode_VfMat\":\"[.9, 1.15, 1.25, 1.5, 1.75, 2.17, 2.6, 2.85; .58, .68, .75, 1.1, 1.38, 1.77, 2.27, 2.7]\",\"diode_VfMat_unit\":\"V\",\"diode_VfMat_conf\":\"compiletime\",\"diode_TjVec\":\"[25, 125]\",\"diode_TjVec_unit\":\"degC\",\"diode_TjVec_conf\":\"compiletime\",\"diode_VfVec\":\"[.5, .7, .9, 1.3, 1.7, 2.1, 2.5]\",\"diode_VfVec_unit\":\"V\",\"diode_VfVec_conf\":\"compiletime\",\"diode_IfVec\":\"[.1, .2, .5, 1, 2, 4, 7, 10]\",\"diode_IfVec_unit\":\"A\",\"diode_IfVec_conf\":\"compiletime\",\"diode_rec_loss_model\":\"ee.enum.diode.reverseRecoveryModel.fixed\",\"diode_rec_loss_model_unit\":\"1\",\"diode_rec_loss_model_conf\":\"compiletime\",\"diode_ErecVal\":\"0\",\"diode_ErecVal_unit\":\"J\",\"diode_ErecVal_conf\":\"compiletime\",\"diode_scaleWithIandV\":\"true\",\"diode_scaleWithIandV_unit\":\"1\",\"diode_scaleWithIandV_conf\":\"compiletime\",\"diode_ErecMat\":\"zeros(2, 3)\",\"diode_ErecMat_unit\":\"J\",\"diode_ErecMat_conf\":\"compiletime\",\"diode_TjrecVec\":\"[298.15, 398.15]\",\"diode_TjrecVec_unit\":\"K\",\"diode_TjrecVec_conf\":\"compiletime\",\"diode_IfrecVec\":\"[.1, 1, 10]\",\"diode_IfrecVec_unit\":\"A\",\"diode_IfrecVec_conf\":\"compiletime\",\"diode_IrecVal\":\"10\",\"diode_IrecVal_unit\":\"A\",\"diode_IrecVal_conf\":\"compiletime\",\"diode_VrecVal\":\"10\",\"diode_VrecVal_unit\":\"V\",\"diode_VrecVal_conf\":\"compiletime\",\"diode_tFilter\":\"1 / 1000 / 100\",\"diode_tFilter_unit\":\"s\",\"diode_tFilter_conf\":\"compiletime\",\"thermal_network_parameterization\":\"ee.enum.thermalNetworkTopology.junctionCase\",\"thermal_network_parameterization_unit\":\"1\",\"thermal_network_parameterization_conf\":\"compiletime\",\"Rth\":\"[0, 10]\",\"Rth_unit\":\"K/W\",\"Rth_conf\":\"compiletime\",\"Rth_Cauer\":\"[1, 3, 10]\",\"Rth_Cauer_unit\":\"K/W\",\"Rth_Cauer_conf\":\"compiletime\",\"Rth_Foster\":\"[.08, .14, .22, .16]\",\"Rth_Foster_unit\":\"K/W\",\"Rth_Foster_conf\":\"compiletime\",\"thermal_mass_parameterization\":\"ee.enum.thermalNetwork.timeconstant\",\"thermal_mass_parameterization_unit\":\"1\",\"thermal_mass_parameterization_conf\":\"compiletime\",\"thermal_mass\":\"[0, 1]\",\"thermal_mass_unit\":\"J/K\",\"thermal_mass_conf\":\"compiletime\",\"thermal_mass_Cauer\":\"[.1, .3, 1]\",\"thermal_mass_Cauer_unit\":\"J/K\",\"thermal_mass_Cauer_conf\":\"compiletime\",\"thermal_mass_Foster\":\"[.001, .005, .05, .5]\",\"thermal_mass_Foster_unit\":\"J/K\",\"thermal_mass_Foster_conf\":\"compiletime\",\"thermal_time_constant\":\"[0, 10]\",\"thermal_time_constant_unit\":\"s\",\"thermal_time_constant_conf\":\"compiletime\",\"thermal_time_constant_Cauer\":\"[1, 3, 10]\",\"thermal_time_constant_Cauer_unit\":\"s\",\"thermal_time_constant_Cauer_conf\":\"compiletime\",\"thermal_time_constant_Foster\":\"[7e-05, .0007, .01, .08]\",\"thermal_time_constant_Foster_unit\":\"s\",\"thermal_time_constant_Foster_conf\":\"compiletime\",\"thermal_mass_initial_temperatures\":\"[25, 25]\",\"thermal_mass_initial_temperatures_unit\":\"degC\",\"thermal_mass_initial_temperatures_conf\":\"compiletime\",\"thermal_mass_initial_temperatures_Cauer\":\"[25, 25, 25]\",\"thermal_mass_initial_temperatures_Cauer_unit\":\"degC\",\"thermal_mass_initial_temperatures_Cauer_conf\":\"compiletime\",\"junction_thermal_mass\":\"0.01\",\"junction_thermal_mass_unit\":\"J/K\",\"junction_thermal_mass_conf\":\"compiletime\",\"Tvec_initial_Foster\":\"[25, 25, 25, 25]\",\"Tvec_initial_Foster_unit\":\"degC\",\"Tvec_initial_Foster_conf\":\"compiletime\",\"junction_temperature_specify\":\"off\",\"junction_temperature_priority\":\"None\",\"junction_temperature\":\"25\",\"junction_temperature_unit\":\"degC\",\"junction_temperature_nominal_specify\":\"off\",\"junction_temperature_nominal_value\":\"1\",\"junction_temperature_nominal_unit\":\"degC\",\"Qj_specify\":\"off\",\"Qj_priority\":\"None\",\"Qj\":\"0\",\"Qj_unit\":\"W\",\"Qj_nominal_specify\":\"off\",\"Qj_nominal_value\":\"1\",\"Qj_nominal_unit\":\"W\",\"accumulatedSwitchingLosses_specify\":\"off\",\"accumulatedSwitchingLosses_priority\":\"None\",\"accumulatedSwitchingLosses\":\"0\",\"accumulatedSwitchingLosses_unit\":\"J\",\"i_H\":\"1\",\"i_H_unit\":\"mA\",\"i_H_conf\":\"compiletime\",\"ia\":\"0\",\"ia_unit\":\"A\",\"ia_specify\":\"off\",\"ia_priority\":\"None\",\"ia_nominal_value\":\"1\",\"ia_nominal_unit\":\"A\",\"ia_nominal_specify\":\"off\",\"Gain\":\"10\",\"Gain_conf\":\"compiletime\",\"Gain_unit\":\"1\",\"IDRM\":\"0.01\",\"IDRM_conf\":\"compiletime\",\"IDRM_unit\":\"mA\",\"IT_vec\":\"[.015, .22, .75, 1.4, 2, 2.75, 3.45]\",\"IT_vec_conf\":\"compiletime\",\"IT_vec_unit\":\"A\",\"Q_npn_bc\":\"0\",\"Q_npn_bc_nominal_specify\":\"off\",\"Q_npn_bc_nominal_unit\":\"uC\",\"Q_npn_bc_nominal_value\":\"1\",\"Q_npn_bc_priority\":\"High\",\"Q_npn_bc_specify\":\"off\",\"Q_npn_bc_unit\":\"C\",\"Q_npn_be\":\"0\",\"Q_npn_be_nominal_specify\":\"off\",\"Q_npn_be_nominal_unit\":\"uC\",\"Q_npn_be_nominal_value\":\"1\",\"Q_npn_be_priority\":\"High\",\"Q_npn_be_specify\":\"off\",\"Q_npn_be_unit\":\"C\",\"Q_pnp_be\":\"0\",\"Q_pnp_be_nominal_specify\":\"off\",\"Q_pnp_be_nominal_unit\":\"uC\",\"Q_pnp_be_nominal_value\":\"1\",\"Q_pnp_be_priority\":\"High\",\"Q_pnp_be_specify\":\"off\",\"Q_pnp_be_unit\":\"C\",\"R\":\"120\",\"R_GK\":\"1000\",\"R_GK_conf\":\"compiletime\",\"R_GK_unit\":\"Ohm\",\"R_conf\":\"compiletime\",\"R_unit\":\"Ohm\",\"Rgate\":\"10\",\"Rgate_conf\":\"compiletime\",\"Rgate_unit\":\"Ohm\",\"Rs\":\"87\",\"Rs_conf\":\"compiletime\",\"Rs_unit\":\"kOhm\",\"TF_NPN\":\"0.3\",\"TF_NPN_conf\":\"compiletime\",\"TF_NPN_parameterization\":\"1\",\"TF_NPN_parameterization_conf\":\"compiletime\",\"TF_NPN_parameterization_unit\":\"1\",\"TF_NPN_unit\":\"us\",\"TF_PNP\":\"0.3\",\"TF_PNP_conf\":\"compiletime\",\"TF_PNP_parameterization\":\"1\",\"TF_PNP_parameterization_conf\":\"compiletime\",\"TF_PNP_parameterization_unit\":\"1\",\"TF_PNP_unit\":\"us\",\"T_d\":\"2\",\"T_d_conf\":\"compiletime\",\"T_d_unit\":\"us\",\"Tmeas\":\"25\",\"Tmeas_conf\":\"compiletime\",\"Tmeas_unit\":\"degC\",\"VDRM\":\"400\",\"VDRM_conf\":\"compiletime\",\"VDRM_unit\":\"V\",\"VT_vec\":\"[.75, 1, 1.25, 1.5, 1.75, 2, 2.25]\",\"VT_vec_conf\":\"compiletime\",\"VT_vec_unit\":\"V\",\"V_D\":\"12\",\"V_D_conf\":\"compiletime\",\"V_D_unit\":\"V\",\"dVdt\":\"150\",\"dVdt_conf\":\"compiletime\",\"dVdt_unit\":\"V/us\",\"i_GT\":\"3\",\"i_GT_conf\":\"compiletime\",\"i_GT_unit\":\"uA\",\"i_d\":\"10\",\"i_d_conf\":\"compiletime\",\"i_d_unit\":\"mA\",\"i_on\":\"1\",\"i_on_conf\":\"compiletime\",\"i_on_unit\":\"A\",\"ig\":\"0\",\"ig_nominal_specify\":\"off\",\"ig_nominal_unit\":\"A\",\"ig_nominal_value\":\"1\",\"ig_priority\":\"None\",\"ig_specify\":\"off\",\"ig_unit\":\"A\",\"model_type\":\"ee.enum.semiconductors.thyristorModelType.equations\",\"model_type_conf\":\"compiletime\",\"model_type_unit\":\"1\",\"t_on_curr\":\"1\",\"t_on_curr_conf\":\"compiletime\",\"t_on_curr_unit\":\"mA\",\"t_on_delay\":\"0\",\"t_on_delay_conf\":\"compiletime\",\"t_on_delay_unit\":\"s\",\"t_on_rise\":\"0\",\"t_on_rise_conf\":\"compiletime\",\"t_on_rise_unit\":\"s\",\"v_GT\":\"0.6\",\"v_GT_conf\":\"compiletime\",\"v_GT_unit\":\"V\",\"v_on\":\"1.2\",\"v_on_conf\":\"compiletime\",\"v_on_unit\":\"V\"}","GTO":""}, Version=25.1, SimscapeInternalDisableModelingOption=on}
      mask prompts: SwitchType "physmod:ee:selector:SwitchingDevice"; LibraryBlockName "physmod:ee:selector:LibraryBlock"; ModelingOption "physmod:ee:selector:ModellingOption"; paramTerminal "physmod:ee:selector:Terminals"; port_option "physmod:ee:selector:PortOption"
      mask help: physmod:ee:selector:SemiconductorSwitch_MD
      settings: CopyFcn=ee.selector.SwitchSelectorUtils.copyCallback
      mask Help: web([docroot '/sps/ref/semiconductorswitchselector.html'])
      mask TypeOptions SwitchType: physmod:ee:selector:MOSFET_PV | physmod:ee:selector:IGBT_PV | physmod:ee:selector:Thyristor_PV | physmod:ee:selector:GTO_PV
      mask Callback SwitchType: ee.selector.SwitchSelectorUtils.selectSwitch
      mask TypeOptions LibraryBlockName: Thyristor | Thyristor (Piecewise Linear)
      mask Callback LibraryBlockName: ee.selector.SwitchSelectorUtils.selectSwitch
      mask TypeOptions ModelingOption: No thermal port | Show thermal port
      mask Callback ModelingOption: ee.selector.SwitchSelectorUtils.selectSwitch
      mask TypeOptions paramTerminal: physmod:ee:library:comments:enum:mosfet:numberOfTerminals:map_Three | physmod:ee:library:comments:enum:mosfet:numberOfTerminals:map_Four
      mask Callback paramTerminal: ee.selector.SwitchSelectorUtils.addOrRemoveFourthPort
      mask TypeOptions port_option: physmod:ee:library:comments:enum:controlport:map_PS | physmod:ee:library:comments:enum:controlport:map_Electrical
      mask Callback port_option: ee.selector.SwitchSelectorUtils.updatePortOption
      mask DialogControl DropdownsTab Prompt: physmod:ee:selector:SwitchSelection
      mask DialogControl SwitchType Prompt: Switching device
      mask DialogControl LibraryBlockName Prompt: Library block
      mask DialogControl ModelingOption Prompt: Modeling option
      mask DialogControl paramTerminal Prompt: Number of terminals
      mask DialogControl port_option Prompt: Gate-control port
      mask DialogControl ConfigureSwitchButton Prompt: physmod:ee:selector:EditParams
      mask DialogControl ConfigureSwitchButton Callback: ee.selector.SwitchSelectorUtils.openSwitchBlock
      mask DialogControl SwitchDescription Prompt: physmod:ee:library:comments:semiconductors:ideal:thyristor:Description
      mask DialogControl RemoveMask Prompt: physmod:ee:selector:RemoveMask
      mask DialogControl RemoveMask Callback: ee.selector.SwitchSelectorUtils.removeMask
  SCR4 : Subsystem  LoadFcn=ee.selector.SwitchSelectorUtils.forwardingCallback  mask(Semiconductor Switch Selector){SwitchType=Thyristor, LibraryBlockName=Thyristor (Piecewise Linear), ModelingOption=No thermal port, ModelingOptionSSCFile=ee.semiconductors.ideal.thyristor, paramTerminal=Three, port_option=Electrical, CachedInstanceParameters=, FormerSwitchType=Thyristor, FormerLibraryBlockName=Thyristor (Piecewise Linear), FormerModelingOption=No thermal port, CachedSharedParameters={"MOSFET":"{\"port_option\":\"ee.enum.controlport.ps\",\"port_option_unit\":\"1\",\"port_option_conf\":\"compiletime\",\"Ron\":\"0.001\",\"Ron_unit\":\"Ohm\",\"Ron_conf\":\"compiletime\",\"Goff\":\"1e-6\",\"Goff_unit\":\"1/Ohm\",\"Goff_conf\":\"compiletime\",\"Vth\":\"0.5\",\"Vth_unit\":\"V\",\"Vth_conf\":\"compiletime\",\"diode_param\":\"ee.enum.semiconductors.protectionDiode.external\",\"diode_param_unit\":\"1\",\"diode_param_conf\":\"compiletime\",\"diode_Vf\":\"0.8\",\"diode_Vf_unit\":\"V\",\"diode_Vf_conf\":\"compiletime\",\"diode_Ron\":\"0.001\",\"diode_Ron_unit\":\"Ohm\",\"diode_Ron_conf\":\"compiletime\",\"diode_Goff\":\"1e-5\",\"diode_Goff_unit\":\"1/Ohm\",\"diode_Goff_conf\":\"compiletime\",\"diode_C\":\"50e-9\",\"diode_C_unit\":\"F\",\"diode_C_conf\":\"compiletime\",\"diode_iRM\":\"-235\",\"diode_iRM_unit\":\"A\",\"diode_iRM_conf\":\"compiletime\",\"diode_iF\":\"300\",\"diode_iF_unit\":\"A\",\"diode_iF_conf\":\"compiletime\",\"diode_idot\":\"-50\",\"diode_idot_unit\":\"A/us\",\"diode_idot_conf\":\"compiletime\",\"diode_trr_param\":\"ee.enum.converters.diodetrr.trr_factor\",\"diode_trr_param_unit\":\"1\",\"diode_trr_param_conf\":\"compiletime\",\"diode_trr_factor\":\"3\",\"diode_trr_factor_unit\":\"1\",\"diode_trr_factor_conf\":\"compiletime\",\"diode_trr\":\"15\",\"diode_trr_unit\":\"us\",\"diode_trr_conf\":\"compiletime\",\"diode_Qrr\":\"1500\",\"diode_Qrr_unit\":\"s*uA\",\"diode_Qrr_conf\":\"compiletime\"}","IGBT":"","Thyristor":"{\"port_option\":\"ee.enum.controlport.elec\",\"port_option_unit\":\"1\",\"port_option_conf\":\"compiletime\",\"Vf\":\"0.8\",\"Vf_unit\":\"V\",\"Vf_conf\":\"compiletime\",\"Ron\":\"0.001\",\"Ron_unit\":\"Ohm\",\"Ron_conf\":\"compiletime\",\"Goff\":\"1e-5\",\"Goff_unit\":\"1/Ohm\",\"Goff_conf\":\"compiletime\",\"Vgt\":\"6\",\"Vgt_unit\":\"V\",\"Vgt_conf\":\"compiletime\",\"diode_param\":\"ee.enum.semiconductors.protectionDiode.external\",\"diode_param_unit\":\"1\",\"diode_param_conf\":\"compiletime\",\"diode_Vf\":\"0.8\",\"diode_Vf_unit\":\"V\",\"diode_Vf_conf\":\"compiletime\",\"diode_Ron\":\"0.001\",\"diode_Ron_unit\":\"Ohm\",\"diode_Ron_conf\":\"compiletime\",\"diode_Goff\":\"1e-5\",\"diode_Goff_unit\":\"1/Ohm\",\"diode_Goff_conf\":\"compiletime\",\"diode_C\":\"50e-9\",\"diode_C_unit\":\"F\",\"diode_C_conf\":\"compiletime\",\"diode_iRM\":\"-235\",\"diode_iRM_unit\":\"A\",\"diode_iRM_conf\":\"compiletime\",\"diode_iF\":\"300\",\"diode_iF_unit\":\"A\",\"diode_iF_conf\":\"compiletime\",\"diode_idot\":\"-50\",\"diode_idot_unit\":\"A/us\",\"diode_idot_conf\":\"compiletime\",\"diode_trr_param\":\"ee.enum.converters.diodetrr.trr_factor\",\"diode_trr_param_unit\":\"1\",\"diode_trr_param_conf\":\"compiletime\",\"diode_trr_factor\":\"3\",\"diode_trr_factor_unit\":\"1\",\"diode_trr_factor_conf\":\"compiletime\",\"diode_trr\":\"15\",\"diode_trr_unit\":\"us\",\"diode_trr_conf\":\"compiletime\",\"diode_Qrr\":\"1500\",\"diode_Qrr_unit\":\"s*uA\",\"diode_Qrr_conf\":\"compiletime\",\"vak_specify\":\"off\",\"vak_priority\":\"None\",\"vak\":\"0\",\"vak_unit\":\"V\",\"vak_nominal_specify\":\"off\",\"vak_nominal_value\":\"1\",\"vak_nominal_unit\":\"V\",\"vgk_specify\":\"off\",\"vgk_priority\":\"None\",\"vgk\":\"0\",\"vgk_unit\":\"V\",\"vgk_nominal_specify\":\"off\",\"vgk_nominal_value\":\"1\",\"vgk_nominal_unit\":\"V\",\"thermal_loss_option\":\"ee.enum.converters.thermalLossOption.constantvalues\",\"thermal_loss_option_unit\":\"1\",\"thermal_loss_option_conf\":\"compiletime\",\"Von_data\":\"[0, .1, .6, .8, 1, 1.3, 1.6, 2, 2.4; 0, .1, .7, 1, 1.2, 1.5, 1.9, 2.4, 2.8]\",\"Von_data_unit\":\"V\",\"Von_data_conf\":\"compiletime\",\"Tj\":\"[298.15, 398.15]\",\"Tj_unit\":\"K\",\"Tj_conf\":\"compiletime\",\"Iout_data\":\"[0, .1, 1, 5, 10, 20, 40, 70, 100]\",\"Iout_data_unit\":\"A\",\"Iout_data_conf\":\"compiletime\",\"Eon_data\":\"[0, .0024, .024, .12, .2, .48, 1.04, 2.16, 3.24; 0, .003, .03, .15, .25, .6, 1.3, 2.7, 4.05] * 1e-3\",\"Eon_data_unit\":\"J\",\"Eon_data_conf\":\"compiletime\",\"Tj_loss\":\"[298.15, 398.15]\",\"Tj_loss_unit\":\"K\",\"Tj_loss_conf\":\"compiletime\",\"Iout_data_loss\":\"[0, .1, 1, 5, 10, 20, 40, 70, 100]\",\"Iout_data_loss_unit\":\"A\",\"Iout_data_loss_conf\":\"compiletime\",\"Eon_scalar\":\"22.86e-3\",\"Eon_scalar_unit\":\"J\",\"Eon_scalar_conf\":\"compiletime\",\"Eoff_natural_commutation\":\"10e-3\",\"Eoff_natural_commutation_unit\":\"J\",\"Eoff_natural_commutation_conf\":\"compiletime\",\"Voff\":\"300\",\"Voff_unit\":\"V\",\"Voff_conf\":\"compiletime\",\"Iout_scalar\":\"600\",\"Iout_scalar_unit\":\"A\",\"Iout_scalar_conf\":\"compiletime\",\"onCurrentMeasDelay\":\"1e-4\",\"onCurrentMeasDelay_unit\":\"s\",\"onCurrentMeasDelay_conf\":\"compiletime\",\"diodeModelType\":\"ee.enum.converters.diodeModelType.pwl\",\"diodeModelType_unit\":\"1\",\"diodeModelType_conf\":\"compiletime\",\"diodeTableType\":\"ee.enum.diode.tableType.IfMat\",\"diodeTableType_unit\":\"1\",\"diodeTableType_conf\":\"compiletime\",\"diode_IfMat\":\"[.07, .12, .19, 1.75, 4.24, 7.32, 11.2; .16, .3, .72, 2.14, 4.02, 6.35, 9.12]\",\"diode_IfMat_unit\":\"A\",\"diode_IfMat_conf\":\"compiletime\",\"diode_VfMat\":\"[.9, 1.15, 1.25, 1.5, 1.75, 2.17, 2.6, 2.85; .58, .68, .75, 1.1, 1.38, 1.77, 2.27, 2.7]\",\"diode_VfMat_unit\":\"V\",\"diode_VfMat_conf\":\"compiletime\",\"diode_TjVec\":\"[25, 125]\",\"diode_TjVec_unit\":\"degC\",\"diode_TjVec_conf\":\"compiletime\",\"diode_VfVec\":\"[.5, .7, .9, 1.3, 1.7, 2.1, 2.5]\",\"diode_VfVec_unit\":\"V\",\"diode_VfVec_conf\":\"compiletime\",\"diode_IfVec\":\"[.1, .2, .5, 1, 2, 4, 7, 10]\",\"diode_IfVec_unit\":\"A\",\"diode_IfVec_conf\":\"compiletime\",\"diode_rec_loss_model\":\"ee.enum.diode.reverseRecoveryModel.fixed\",\"diode_rec_loss_model_unit\":\"1\",\"diode_rec_loss_model_conf\":\"compiletime\",\"diode_ErecVal\":\"0\",\"diode_ErecVal_unit\":\"J\",\"diode_ErecVal_conf\":\"compiletime\",\"diode_scaleWithIandV\":\"true\",\"diode_scaleWithIandV_unit\":\"1\",\"diode_scaleWithIandV_conf\":\"compiletime\",\"diode_ErecMat\":\"zeros(2, 3)\",\"diode_ErecMat_unit\":\"J\",\"diode_ErecMat_conf\":\"compiletime\",\"diode_TjrecVec\":\"[298.15, 398.15]\",\"diode_TjrecVec_unit\":\"K\",\"diode_TjrecVec_conf\":\"compiletime\",\"diode_IfrecVec\":\"[.1, 1, 10]\",\"diode_IfrecVec_unit\":\"A\",\"diode_IfrecVec_conf\":\"compiletime\",\"diode_IrecVal\":\"10\",\"diode_IrecVal_unit\":\"A\",\"diode_IrecVal_conf\":\"compiletime\",\"diode_VrecVal\":\"10\",\"diode_VrecVal_unit\":\"V\",\"diode_VrecVal_conf\":\"compiletime\",\"diode_tFilter\":\"1 / 1000 / 100\",\"diode_tFilter_unit\":\"s\",\"diode_tFilter_conf\":\"compiletime\",\"thermal_network_parameterization\":\"ee.enum.thermalNetworkTopology.junctionCase\",\"thermal_network_parameterization_unit\":\"1\",\"thermal_network_parameterization_conf\":\"compiletime\",\"Rth\":\"[0, 10]\",\"Rth_unit\":\"K/W\",\"Rth_conf\":\"compiletime\",\"Rth_Cauer\":\"[1, 3, 10]\",\"Rth_Cauer_unit\":\"K/W\",\"Rth_Cauer_conf\":\"compiletime\",\"Rth_Foster\":\"[.08, .14, .22, .16]\",\"Rth_Foster_unit\":\"K/W\",\"Rth_Foster_conf\":\"compiletime\",\"thermal_mass_parameterization\":\"ee.enum.thermalNetwork.timeconstant\",\"thermal_mass_parameterization_unit\":\"1\",\"thermal_mass_parameterization_conf\":\"compiletime\",\"thermal_mass\":\"[0, 1]\",\"thermal_mass_unit\":\"J/K\",\"thermal_mass_conf\":\"compiletime\",\"thermal_mass_Cauer\":\"[.1, .3, 1]\",\"thermal_mass_Cauer_unit\":\"J/K\",\"thermal_mass_Cauer_conf\":\"compiletime\",\"thermal_mass_Foster\":\"[.001, .005, .05, .5]\",\"thermal_mass_Foster_unit\":\"J/K\",\"thermal_mass_Foster_conf\":\"compiletime\",\"thermal_time_constant\":\"[0, 10]\",\"thermal_time_constant_unit\":\"s\",\"thermal_time_constant_conf\":\"compiletime\",\"thermal_time_constant_Cauer\":\"[1, 3, 10]\",\"thermal_time_constant_Cauer_unit\":\"s\",\"thermal_time_constant_Cauer_conf\":\"compiletime\",\"thermal_time_constant_Foster\":\"[7e-05, .0007, .01, .08]\",\"thermal_time_constant_Foster_unit\":\"s\",\"thermal_time_constant_Foster_conf\":\"compiletime\",\"thermal_mass_initial_temperatures\":\"[25, 25]\",\"thermal_mass_initial_temperatures_unit\":\"degC\",\"thermal_mass_initial_temperatures_conf\":\"compiletime\",\"thermal_mass_initial_temperatures_Cauer\":\"[25, 25, 25]\",\"thermal_mass_initial_temperatures_Cauer_unit\":\"degC\",\"thermal_mass_initial_temperatures_Cauer_conf\":\"compiletime\",\"junction_thermal_mass\":\"0.01\",\"junction_thermal_mass_unit\":\"J/K\",\"junction_thermal_mass_conf\":\"compiletime\",\"Tvec_initial_Foster\":\"[25, 25, 25, 25]\",\"Tvec_initial_Foster_unit\":\"degC\",\"Tvec_initial_Foster_conf\":\"compiletime\",\"junction_temperature_specify\":\"off\",\"junction_temperature_priority\":\"None\",\"junction_temperature\":\"25\",\"junction_temperature_unit\":\"degC\",\"junction_temperature_nominal_specify\":\"off\",\"junction_temperature_nominal_value\":\"1\",\"junction_temperature_nominal_unit\":\"degC\",\"Qj_specify\":\"off\",\"Qj_priority\":\"None\",\"Qj\":\"0\",\"Qj_unit\":\"W\",\"Qj_nominal_specify\":\"off\",\"Qj_nominal_value\":\"1\",\"Qj_nominal_unit\":\"W\",\"accumulatedSwitchingLosses_specify\":\"off\",\"accumulatedSwitchingLosses_priority\":\"None\",\"accumulatedSwitchingLosses\":\"0\",\"accumulatedSwitchingLosses_unit\":\"J\",\"i_H\":\"1\",\"i_H_unit\":\"mA\",\"i_H_conf\":\"compiletime\",\"ia\":\"0\",\"ia_unit\":\"A\",\"ia_specify\":\"off\",\"ia_priority\":\"None\",\"ia_nominal_value\":\"1\",\"ia_nominal_unit\":\"A\",\"ia_nominal_specify\":\"off\",\"Gain\":\"10\",\"Gain_conf\":\"compiletime\",\"Gain_unit\":\"1\",\"IDRM\":\"0.01\",\"IDRM_conf\":\"compiletime\",\"IDRM_unit\":\"mA\",\"IT_vec\":\"[.015, .22, .75, 1.4, 2, 2.75, 3.45]\",\"IT_vec_conf\":\"compiletime\",\"IT_vec_unit\":\"A\",\"Q_npn_bc\":\"0\",\"Q_npn_bc_nominal_specify\":\"off\",\"Q_npn_bc_nominal_unit\":\"uC\",\"Q_npn_bc_nominal_value\":\"1\",\"Q_npn_bc_priority\":\"High\",\"Q_npn_bc_specify\":\"off\",\"Q_npn_bc_unit\":\"C\",\"Q_npn_be\":\"0\",\"Q_npn_be_nominal_specify\":\"off\",\"Q_npn_be_nominal_unit\":\"uC\",\"Q_npn_be_nominal_value\":\"1\",\"Q_npn_be_priority\":\"High\",\"Q_npn_be_specify\":\"off\",\"Q_npn_be_unit\":\"C\",\"Q_pnp_be\":\"0\",\"Q_pnp_be_nominal_specify\":\"off\",\"Q_pnp_be_nominal_unit\":\"uC\",\"Q_pnp_be_nominal_value\":\"1\",\"Q_pnp_be_priority\":\"High\",\"Q_pnp_be_specify\":\"off\",\"Q_pnp_be_unit\":\"C\",\"R\":\"120\",\"R_GK\":\"1000\",\"R_GK_conf\":\"compiletime\",\"R_GK_unit\":\"Ohm\",\"R_conf\":\"compiletime\",\"R_unit\":\"Ohm\",\"Rgate\":\"10\",\"Rgate_conf\":\"compiletime\",\"Rgate_unit\":\"Ohm\",\"Rs\":\"87\",\"Rs_conf\":\"compiletime\",\"Rs_unit\":\"kOhm\",\"TF_NPN\":\"0.3\",\"TF_NPN_conf\":\"compiletime\",\"TF_NPN_parameterization\":\"1\",\"TF_NPN_parameterization_conf\":\"compiletime\",\"TF_NPN_parameterization_unit\":\"1\",\"TF_NPN_unit\":\"us\",\"TF_PNP\":\"0.3\",\"TF_PNP_conf\":\"compiletime\",\"TF_PNP_parameterization\":\"1\",\"TF_PNP_parameterization_conf\":\"compiletime\",\"TF_PNP_parameterization_unit\":\"1\",\"TF_PNP_unit\":\"us\",\"T_d\":\"2\",\"T_d_conf\":\"compiletime\",\"T_d_unit\":\"us\",\"Tmeas\":\"25\",\"Tmeas_conf\":\"compiletime\",\"Tmeas_unit\":\"degC\",\"VDRM\":\"400\",\"VDRM_conf\":\"compiletime\",\"VDRM_unit\":\"V\",\"VT_vec\":\"[.75, 1, 1.25, 1.5, 1.75, 2, 2.25]\",\"VT_vec_conf\":\"compiletime\",\"VT_vec_unit\":\"V\",\"V_D\":\"12\",\"V_D_conf\":\"compiletime\",\"V_D_unit\":\"V\",\"dVdt\":\"150\",\"dVdt_conf\":\"compiletime\",\"dVdt_unit\":\"V/us\",\"i_GT\":\"3\",\"i_GT_conf\":\"compiletime\",\"i_GT_unit\":\"uA\",\"i_d\":\"10\",\"i_d_conf\":\"compiletime\",\"i_d_unit\":\"mA\",\"i_on\":\"1\",\"i_on_conf\":\"compiletime\",\"i_on_unit\":\"A\",\"ig\":\"0\",\"ig_nominal_specify\":\"off\",\"ig_nominal_unit\":\"A\",\"ig_nominal_value\":\"1\",\"ig_priority\":\"None\",\"ig_specify\":\"off\",\"ig_unit\":\"A\",\"model_type\":\"ee.enum.semiconductors.thyristorModelType.equations\",\"model_type_conf\":\"compiletime\",\"model_type_unit\":\"1\",\"t_on_curr\":\"1\",\"t_on_curr_conf\":\"compiletime\",\"t_on_curr_unit\":\"mA\",\"t_on_delay\":\"0\",\"t_on_delay_conf\":\"compiletime\",\"t_on_delay_unit\":\"s\",\"t_on_rise\":\"0\",\"t_on_rise_conf\":\"compiletime\",\"t_on_rise_unit\":\"s\",\"v_GT\":\"0.6\",\"v_GT_conf\":\"compiletime\",\"v_GT_unit\":\"V\",\"v_on\":\"1.2\",\"v_on_conf\":\"compiletime\",\"v_on_unit\":\"V\"}","GTO":""}, Version=25.1, SimscapeInternalDisableModelingOption=on}
      mask prompts: SwitchType "physmod:ee:selector:SwitchingDevice"; LibraryBlockName "physmod:ee:selector:LibraryBlock"; ModelingOption "physmod:ee:selector:ModellingOption"; paramTerminal "physmod:ee:selector:Terminals"; port_option "physmod:ee:selector:PortOption"
      mask help: physmod:ee:selector:SemiconductorSwitch_MD
      settings: CopyFcn=ee.selector.SwitchSelectorUtils.copyCallback
      mask Help: web([docroot '/sps/ref/semiconductorswitchselector.html'])
      mask TypeOptions SwitchType: physmod:ee:selector:MOSFET_PV | physmod:ee:selector:IGBT_PV | physmod:ee:selector:Thyristor_PV | physmod:ee:selector:GTO_PV
      mask Callback SwitchType: ee.selector.SwitchSelectorUtils.selectSwitch
      mask TypeOptions LibraryBlockName: Thyristor | Thyristor (Piecewise Linear)
      mask Callback LibraryBlockName: ee.selector.SwitchSelectorUtils.selectSwitch
      mask TypeOptions ModelingOption: No thermal port | Show thermal port
      mask Callback ModelingOption: ee.selector.SwitchSelectorUtils.selectSwitch
      mask TypeOptions paramTerminal: physmod:ee:library:comments:enum:mosfet:numberOfTerminals:map_Three | physmod:ee:library:comments:enum:mosfet:numberOfTerminals:map_Four
      mask Callback paramTerminal: ee.selector.SwitchSelectorUtils.addOrRemoveFourthPort
      mask TypeOptions port_option: physmod:ee:library:comments:enum:controlport:map_PS | physmod:ee:library:comments:enum:controlport:map_Electrical
      mask Callback port_option: ee.selector.SwitchSelectorUtils.updatePortOption
      mask DialogControl DropdownsTab Prompt: physmod:ee:selector:SwitchSelection
      mask DialogControl SwitchType Prompt: Switching device
      mask DialogControl LibraryBlockName Prompt: Library block
      mask DialogControl ModelingOption Prompt: Modeling option
      mask DialogControl paramTerminal Prompt: Number of terminals
      mask DialogControl port_option Prompt: Gate-control port
      mask DialogControl ConfigureSwitchButton Prompt: physmod:ee:selector:EditParams
      mask DialogControl ConfigureSwitchButton Callback: ee.selector.SwitchSelectorUtils.openSwitchBlock
      mask DialogControl SwitchDescription Prompt: physmod:ee:library:comments:semiconductors:ideal:thyristor:Description
      mask DialogControl RemoveMask Prompt: physmod:ee:selector:RemoveMask
      mask DialogControl RemoveMask Callback: ee.selector.SwitchSelectorUtils.removeMask
  Scope : Scope
  Solver Configuration : nesl_utility/Solver Configuration  PhysicalDomain=network_engine_domain  SubClassName=solver  LeftPortType=input  RightPortType=generic  Tones=[]  Harmonics=[]  SimulateNoise=off  Profile=off  UseLocalSampling=off  EnableSwitchedLinearOptims=on  FrequencyDomain=off  UseCCode=off  RelTol=0.001  AbsTol=0.001  MinStep=1e-09  ToWorkspace=off  RevertToSquareIcSolve=off  NumHomotopyIterations=100  PhasorMode=off  PhasorModeNumHarmonics=1  ConsistencySolver=NEWTON_XTOL_AFTER_FTOL  IndexReductionMethod=DerivativeReplacement  DoDC=off  ResidualTolerance=1e-09  ConsistencyTolSource=GLOBAL  ConsistencyAbsTol=0.001  ConsistencyRelTol=0.001  ConsistencyTolFactor=0.001  UseLocalSolver=off  LocalSolverChoice=NE_BACKWARD_EULER_ADVANCER  ResolveIndetEquations=on  FunctionEvalNumThread=1  LocalSolverSampleTime=0.001  DoFixedCost=off  MaxNonlinIter=3  MaxModeIter=2  ComputeImpulses=off  ImpulseIterations=2  LinearAlgebra=auto  LinearAlgebraNumThread=0  EquationFormulation=NE_TIME_EF  DelaysMemoryBudget=1024  AutomaticFiltering=on  FilteringTimeConstant=0.001  PartitionStorageMethod=AS_NEEDED  PartitionMemoryBudget=1024  PartitionMethod=ROBUST  MultibodyUseLocalSolver=off  MultibodyLocalSolverChoice=ODE1  MultibodyLocalSolverSampleTime=0.001
  rpm : Scope
      settings: ActiveDisplayYMinimum=-19822.265966346931  ActiveDisplayYMaximum=38369.115005662679
  wires:
  PS-Simulink Converter4/1 -> Gain/1
  Gain/1 -> SCR gate pulses/5(speed), rpm/1
  Clock/1 -> SCR gate pulses/2(t)
  SCR gate pulses/1(g1) -> Data Type Conversion/1
  SCR gate pulses/4(g4) -> Data Type Conversion3/1
  SCR gate pulses/3(g3) -> Data Type Conversion2/1
  SCR gate pulses/2(g2) -> Data Type Conversion1/1
  Data Type Conversion/1 -> PS1/1
  Data Type Conversion1/1 -> PS2/1
  Data Type Conversion2/1 -> PS3/1
  Data Type Conversion3/1 -> PS4/1
  Constant/1 -> SCR gate pulses/1(u)
  Constant1/1 -> SCR gate pulses/3(alpha)
  Constant2/1 -> SCR gate pulses/4(brake)
  PS-Simulink Converter/1 -> Scope/1
  connections:
  AC Voltage Source/LConn1 -- SCR1/RConn1 -- Controlled Voltage Source1/RConn2 -- SCR3/RConn2
  Controlled Voltage Source2/RConn2 -- SCR2/RConn2 -- DC Motor/LConn2 -- Current Sensor/RConn2
  AC Voltage Source/RConn1 -- Solver Configuration/RConn1 -- Electrical Reference/LConn1 -- SCR4/RConn2 -- Controlled Voltage Source3/RConn2 -- SCR2/RConn1
  SCR3/RConn1 -- DC Motor/RConn2 -- SCR4/RConn1
  Controlled Voltage Source/LConn1 -- Resistor/LConn1
  Resistor/RConn1 -- SCR1/LConn1
  Controlled Voltage Source1/LConn1 -- Resistor1/LConn1
  Resistor1/RConn1 -- SCR3/LConn1
  Controlled Voltage Source2/LConn1 -- Resistor2/LConn1
  Resistor2/RConn1 -- SCR2/LConn1
  Controlled Voltage Source3/LConn1 -- Resistor3/LConn1
  Resistor3/RConn1 -- SCR4/LConn1
  DC Motor/LConn3 -- Ideal Rotational Motion Sensor/LConn1
  DC Motor/RConn3 -- Ideal Rotational Motion Sensor/RConn1 -- Mechanical Rotational Reference/LConn1
  PS-Simulink Converter4/LConn1 -- Ideal Rotational Motion Sensor/RConn2
  PS1/RConn1 -- Controlled Voltage Source/RConn1
  PS2/RConn1 -- Controlled Voltage Source2/RConn1
  PS3/RConn1 -- Controlled Voltage Source1/RConn1
  PS4/RConn1 -- Controlled Voltage Source3/RConn1
  Controlled Voltage Source/RConn2 -- SCR1/RConn2 -- Current Sensor/LConn1
  PS-Simulink Converter/LConn1 -- Current Sensor/RConn1
